simulink model "dyn_control"  (R2022a)
settings: Solver=VariableStepAuto  StartTime=0.0  StopTime=2  FixedStep=0.1  RelTol=1e-2
undefined symbols (not defined in the file): D, E_1, E_2, g, Gs_1, Gs_2, Ia_1, Ia_2, Im_1, Im_2, l_1, l_2, m_1, m_2, q_0, q_dot_0, t1_p, t2_p, t3_p, t4_p, t5_p, twt
libraries: slpidlib x2, matrix_library x2, dspinverses x2
settings Model: Creator=luca  LastModifiedBy=atled
settings SolverCC: AllowMultiTaskInputOutput=on  PositivePriorityOrder=on  AutoInsertRateTranBlk=on
settings HardwareCC: TargetBitPerPointer=64  TargetBitPerSizeT=64  TargetBitPerPtrDiffT=64  TargetLongLongMode=on  TargetIntDivRoundTo=Zero  TargetEndianess=LittleEndian  TargetWordSize=64  TargetHWDeviceType=MATLAB Host  ProdEqTarget=off
settings RTWCC: SystemTargetFile=raccel.tlc  TemplateMakefile=raccel_default_tmf  RTWVerbose=off
settings CodeAppCC: GenerateComments=off  MaxIdLength=128  SimulinkBlockComments=off
settings RaccelTargetCC: TargetLangStandard=C99 (ISO)  OptimizeReductions=off  ENABLE_SLEXEC_SSBRIDGE=1  RTWCAPISignals=off  RTWCAPIParams=off  RTWCAPIRootIO=off

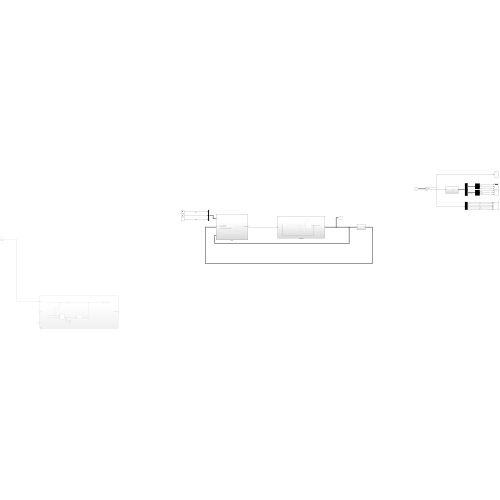
[thumbnail: Simulink's stored preview of the top-level diagram]
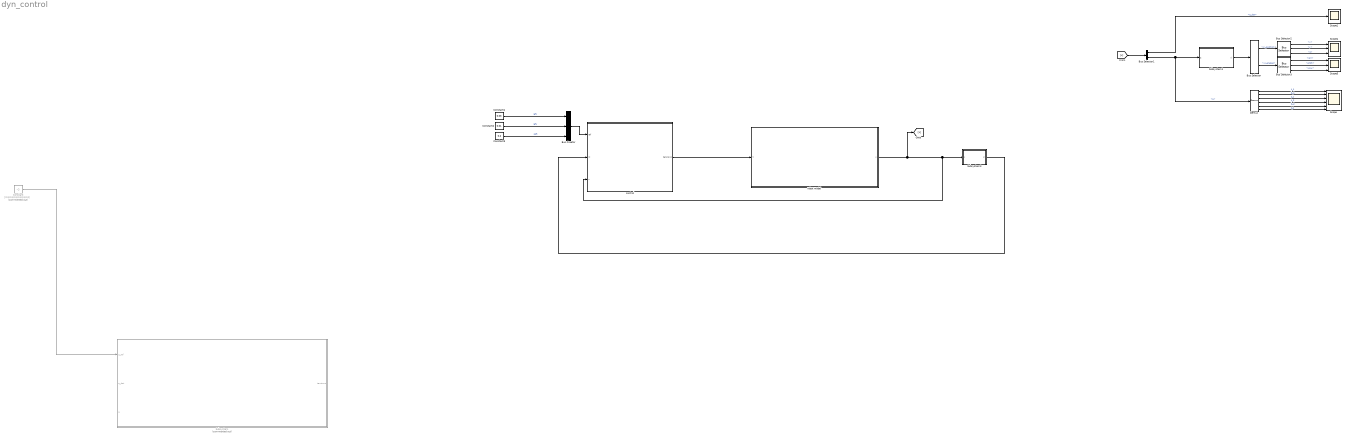
== system dyn_control ==
  Bus Creator : BusCreator  Inputs=3
  Bus Selector : BusSelector  OutputSignals=xi_position,xi_angles
  Bus Selector1 : BusSelector  OutputSignals=q_dot,q
  Bus Selector2 : BusSelector  OutputSignals=x,y,z
  Bus Selector3 : BusSelector  OutputSignals=roll,pitch,yaw
  Constant : Constant  Commented=on  Value=[0.3,0.3,0.3,0.3,0.3,0.3]
  Constant1 : Constant  Value=0.03  VectorParams1D=off
  Constant2 : Constant  Value=0.01  VectorParams1D=off
  Constant3 : Constant  Value=0.2  VectorParams1D=off
  Demux : Demux  Outputs=6
  Scope : Scope  NumInputPorts=6
  Scope1 : Scope
  Scope4 : Scope  NumInputPorts=3
  Scope5 : Scope  NumInputPorts=3
  Subsystem : Subsystem  Commented=on
  Subsystem1 : Subsystem
  Subsystem3 : Subsystem
  control : Subsystem
  robot model : Subsystem
  wires:
  Demux/1 -> Scope/1  "k_1"
  Demux/2 -> Scope/2  "b_1"
  Demux/3 -> Scope/3  "t_1"
  Demux/4 -> Scope/4  "k_2"
  Demux/5 -> Scope/5  "b_2"
  Demux/6 -> Scope/6  "t_2"
  Constant/1 -> Subsystem/1(q_ref)
  Subsystem1/1(xi) -> Bus Selector/1
  Bus Selector/1 -> Bus Selector2/1  "<xi_position>"
  Bus Selector/2 -> Bus Selector3/1  "<xi_angles>"
  [x] -> Bus Selector1/1
  Bus Selector1/2 -> Demux/1, Subsystem1/1(q)  "<q>"
  Bus Selector1/1 -> Scope1/1  "<q_dot>"
  Subsystem3/1(xi) -> control/2(Xi)
  robot model/1(x) -> [x], control/3(x), Subsystem3/1(x)
  Constant1/1 -> Bus Creator/1  "refx"
  Bus Selector2/1 -> Scope4/1  "<x>"
  Bus Selector2/2 -> Scope4/2  "<y>"
  Bus Selector2/3 -> Scope4/3  "<z>"
  Bus Selector3/1 -> Scope5/1  "<roll>"
  Bus Selector3/2 -> Scope5/2  "<pitch>"
  Bus Selector3/3 -> Scope5/3  "<yaw>"
  Constant2/1 -> Bus Creator/2  "refy"
  Constant3/1 -> Bus Creator/3  "refz"
  Bus Creator/1 -> control/1(ref)
  control/1(tensions) -> robot model/1(t)

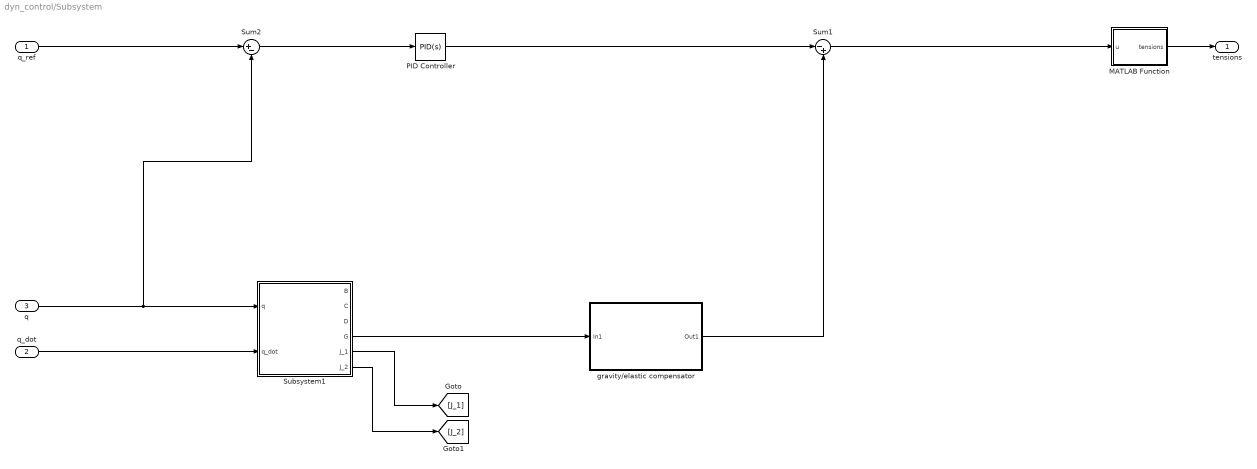
== system dyn_control/Subsystem ==
  q_ref : Inport
  q_dot : Inport  Port=2
  q : Inport  Port=3
  MATLAB Function : MATLAB Function  TreatAsAtomicUnit=on
  PID Controller : slpidlib/PID Controller  Controller=PID  Form=Parallel  TimeDomain=Continuous-time  UseExternalTs=off  SampleTime=-1  IntegratorMethod=Forward Euler  FilterMethod=Forward Euler  ControllerParametersSource=internal  P=1  I=0  UseKiTs=off  D=0.01  N=100  UseFilter=on  TunerSelectOption=Transfer Function Based (PID Tuner App)  InitialConditionSource=internal  InitialConditionForIntegrator=0  InitialConditionForFilter=0  DifferentiatorICPrevScaledInput=0  ExternalReset=none  TrackingMode=off  Kt=1  LimitOutput=off  SatLimitsSource=internal  UpperSaturationLimit=inf  LowerSaturationLimit=-inf  LinearizeAsGain=on  AntiWindupMode=none  Kb=1  POutMin=[]  POutMax=[]  IOutMin=[]  IOutMax=[]  DOutMin=[]  DOutMax=[]  NOutMin=[]  NOutMax=[]  SumOutMin=[]  SumOutMax=[]  SaturationOutMin=[]  SaturationOutMax=[]  PParamMin=[]  PParamMax=[]  IParamMin=[]  IParamMax=[]  DParamMin=[]  DParamMax=[]  NParamMin=[]  NParamMax=[]  KbParamMin=[]  KbParamMax=[]  KtParamMin=[]  KtParamMax=[]  KbOutMin=[]  KbOutMax=[]  KtOutMin=[]  KtOutMax=[]  IntegratorOutMin=[]  IntegratorOutMax=[]  FilterOutMin=[]  FilterOutMax=[]  SumI1OutMin=[]  SumI1OutMax=[]  SumI2OutMin=[]  SumI2OutMax=[]  SumI3OutMin=[]  SumI3OutMax=[]  SumI4OutMin=[]  SumI4OutMax=[]  SumDOutMin=[]  SumDOutMax=[]  DifferentiatorOutMin=[]  DifferentiatorOutMax=[]  FilterDiffOutCoefMin=[]  FilterDiffOutCoefMax=[]  ReciprocalOutMin=[]  ReciprocalOutMax=[]  SumDenOutMin=[]  SumDenOutMax=[]  SumNumOutMin=[]  SumNumOutMax=[]  DivideOutMin=[]  DivideOutMax=[]  UdiffTsProdOutMin=[]  UdiffTsProdOutMax=[]  NTsProdOutMin=[]  NTsProdOutMax=[]  UintegralTsProdOutMin=[]  UintegralTsProdOutMax=[]  UngainTsProdOutMin=[]  UngainTsProdOutMax=[]  IntegratorContinuousStateAttributes=''  IntegratorStateMustResolveToSignalObject=off  IntegratorRTWStateStorageClass=Auto  FilterContinuousStateAttributes=''  FilterStateMustResolveToSignalObject=off  FilterRTWStateStorageClass=Auto  ParallelPVariant=InternalParameters  IdealPVariant=Disabled  IVariant=InternalParameters  DVariant=InternalParameters  IntegratorVariant=Continuous  SatVariant=Disabled  AWVariant=Passthrough  PCopyVariant=Disabled  TRVariant=Disabled  FdbkBlocksVariant=Forward  IdealPFdbkVariant=Disabled  SatFdbkVariant=Disabled  DerivativeFilterVariant=ContFilter  NVariant=InternalParameters  NCopyVariant=Disabled  FilterICVariant=InternalICsFilter  IntegratorICVariant=InternalICs  ExternalResetVariant=Disabled  TRSumVariant=Passthrough  SumFdbkVariant=Disabled  SumVariant=Sum_PID  TsampFilterVariant=InternalTs  TsampNgainVariant=Passthrough  TsampIntegralVariant=Passthrough  ExternalSaturationOutDataTypeStr=Inherit: Same as second input  aMode=0
  Subsystem1 : Subsystem
  Sum1 : Sum  Inputs=|-+
  Sum2 : Sum  Inputs=|+-
  gravity/elastic compensator : Subsystem
  tensions : Outport
  wires:
  q/1 -> Subsystem1/1(q), Sum2/2
  q_dot/1 -> Subsystem1/2(q_dot)
  Subsystem1/4(G) -> gravity/elastic compensator/1(In1)
  gravity/elastic compensator/1(Out1) -> Sum1/2
  q_ref/1 -> Sum2/1
  PID Controller/1 -> Sum1/1
  Sum2/1 -> PID Controller/1
  Sum1/1 -> MATLAB Function/1(u)
  Subsystem1/5(J_1) -> [J_1]
  Subsystem1/6(J_2) -> [J_2]
  MATLAB Function/1(tensions) -> tensions/1

== system dyn_control/Subsystem1 ==
  q : Inport
  Bus Creator : BusCreator  Inputs=3
  Bus Creator1 : BusCreator  Inputs=2
  Bus Creator2 : BusCreator  Inputs=3
  Constant : Constant  Value=l_1
  Constant1 : Constant  Value=l_2
  MATLAB Function1 : MATLAB Function  TreatAsAtomicUnit=on
  xi : Outport
  wires:
  Constant1/1 -> MATLAB Function1/3(l_2)
  q/1 -> MATLAB Function1/1(q)
  Constant/1 -> MATLAB Function1/2(l_1)
  MATLAB Function1/1(x) -> Bus Creator/1  "x"
  MATLAB Function1/2(y) -> Bus Creator/2  "y"
  MATLAB Function1/3(z) -> Bus Creator/3  "z"
  MATLAB Function1/4(roll) -> Bus Creator2/1  "roll"
  MATLAB Function1/5(pitch) -> Bus Creator2/2  "pitch"
  MATLAB Function1/6(yaw) -> Bus Creator2/3  "yaw"
  Bus Creator/1 -> Bus Creator1/1  "xi_position"
  Bus Creator2/1 -> Bus Creator1/2  "xi_angles"
  Bus Creator1/1 -> xi/1

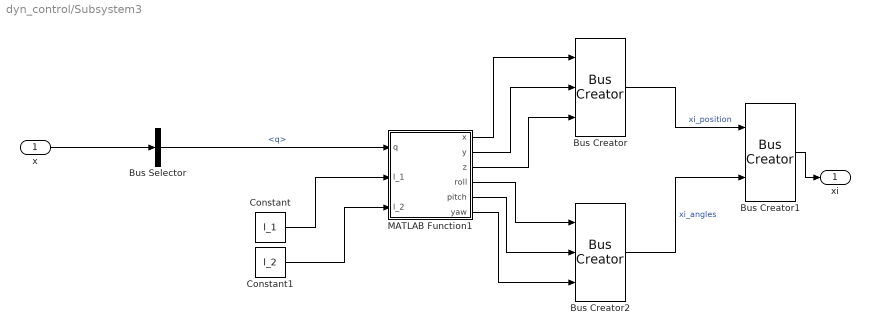
== system dyn_control/Subsystem3 ==
  x : Inport
  Bus Creator : BusCreator  Inputs=3
  Bus Creator1 : BusCreator  Inputs=2
  Bus Creator2 : BusCreator  Inputs=3
  Bus Selector : BusSelector  OutputSignals=q
  Constant : Constant  Value=l_1
  Constant1 : Constant  Value=l_2
  MATLAB Function1 : MATLAB Function  TreatAsAtomicUnit=on
  xi : Outport
  wires:
  Constant1/1 -> MATLAB Function1/3(l_2)
  Constant/1 -> MATLAB Function1/2(l_1)
  MATLAB Function1/1(x) -> Bus Creator/1
  MATLAB Function1/2(y) -> Bus Creator/2
  MATLAB Function1/3(z) -> Bus Creator/3
  MATLAB Function1/4(roll) -> Bus Creator2/1
  MATLAB Function1/5(pitch) -> Bus Creator2/2
  MATLAB Function1/6(yaw) -> Bus Creator2/3
  Bus Creator/1 -> Bus Creator1/1  "xi_position"
  Bus Creator2/1 -> Bus Creator1/2  "xi_angles"
  Bus Creator1/1 -> xi/1
  x/1 -> Bus Selector/1
  Bus Selector/1 -> MATLAB Function1/1(q)  "<q>"

== system dyn_control/control ==
  ref : Inport
  Xi : Inport  Port=2
  x : Inport  Port=3
  PD : Subsystem
      settings: PortSchema="{\"entries\":[{\"content\":{\"sides\":[{\"content\":{\"connectorIds\":[\"In1\",\"In2\"]},\"type\":\"ConnectorPlacement.EquallySpacedRectSide\",\"uuid\":\"ef742de7-f960-40b6-94f7-85e648a2417a\"},{\"content\":{\"connectorIds\":[\"Out1\"],\"side\":\"RIGHT\"},\"type\":\"ConnectorPlacement.EquallySpacedRectSide\",\"uuid\":\"e206da22-0c0c-407f-8f6d-88bececd3830\"},{\"content\":{\"connectorIds\":[],\"side\":\"TOP\"},\"type\":\"ConnectorPlacement.EquallySpacedRectSide\",\"uuid\":\"14c35c5b-992e-4e43-89c3-904fa34ec5bf\"},{\"content\":{\"connectorIds\":[\"In3\"],\"side\":\"BOTTOM\"},\"type\":\"ConnectorPlacement.EquallySpacedRectSide\",\"uuid\":\"998b2191-7e30-46d3-8883-46ecfd785cdd\"}]},\"type\":\"ConnectorPlacement.EquallySpacedConnector\",\"uuid\":\"de184336-5ab9-4a9a-8417-f4954e1c5ad0\"}],\"packageUris\":[\"http://schema.mathworks.com/mf0/Connector/R2020b\"],\"version\":\"1.0\"}"
  tensions : Outport
  wires:
  ref/1 -> PD/1(In1)
  Xi/1 -> PD/2(In2)
  x/1 -> PD/3(x)
  PD/1(t) -> tensions/1

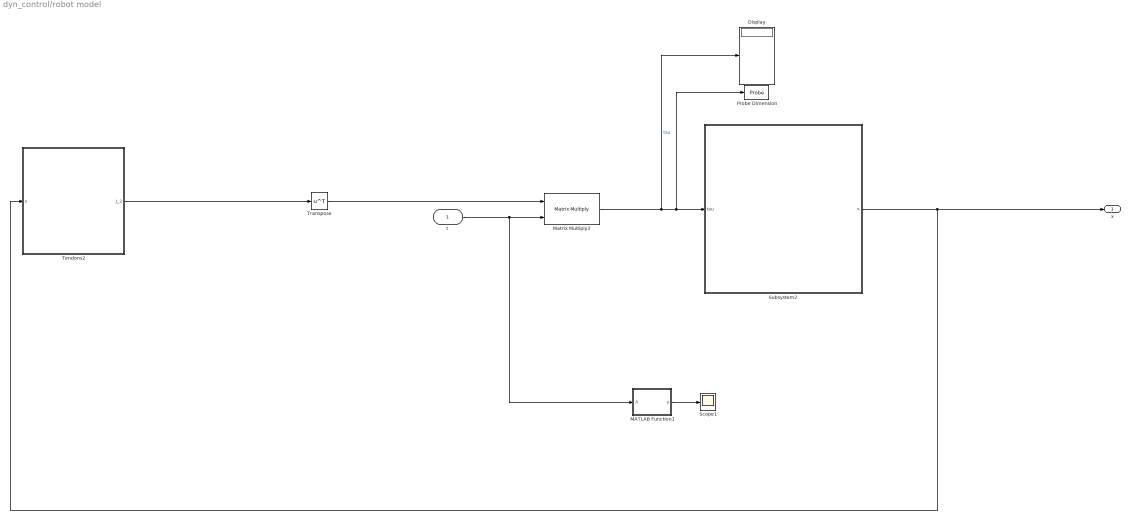
== system dyn_control/robot model ==
  t : Inport
  Display : Display
  MATLAB Function1 : MATLAB Function  TreatAsAtomicUnit=on
  Matrix Multiply3 : Product  Multiplication=Matrix(*)
  Probe Dimension : Probe  ProbeWidth=off  ProbeSampleTime=off  ProbeComplexSignal=off  ProbeSignalDimensions=on
  Scope1 : Scope
  Subsystem2 : Subsystem
  Tendons2 : Subsystem
  Transpose : Math  Operator=transpose
  x : Outport
  wires:
  Subsystem2/1(x) -> Tendons2/1(x), x/1
  Matrix Multiply3/1 -> Display/1, Probe Dimension/1, Subsystem2/1(tau)  "tau"
  Tendons2/1(J_2) -> Transpose/1
  Transpose/1 -> Matrix Multiply3/1
  t/1 -> MATLAB Function1/1(A), Matrix Multiply3/2
  MATLAB Function1/1(y) -> Scope1/1

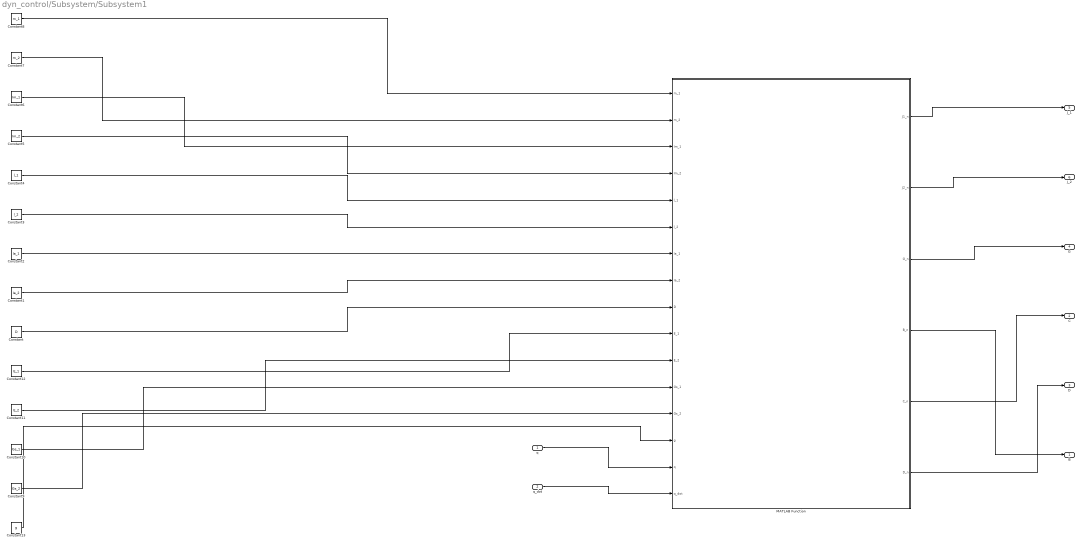
== system dyn_control/Subsystem/Subsystem1 ==
  q : Inport
  q_dot : Inport  Port=2
  Constant : Constant  Value=D
  Constant1 : Constant  Value=Ia_2
  Constant10 : Constant  Value=Gs_1
  Constant11 : Constant  Value=E_2
  Constant12 : Constant  Value=E_1
  Constant13 : Constant  Value=g
  Constant2 : Constant  Value=Ia_1
  Constant3 : Constant  Value=l_2
  Constant4 : Constant  Value=l_1
  Constant5 : Constant  Value=Im_2
  Constant6 : Constant  Value=Im_1
  Constant7 : Constant  Value=m_2
  Constant8 : Constant  Value=m_1
  Constant9 : Constant  Value=Gs_2
  MATLAB Function : MATLAB Function  TreatAsAtomicUnit=on
  B : Outport
  C : Outport  Port=2
  D : Outport  Port=3
  G : Outport  Port=4
  J_1 : Outport  Port=5
  J_2 : Outport  Port=6
  wires:
  MATLAB Function/1(J1_n) -> J_1/1
  MATLAB Function/3(G_n) -> G/1
  MATLAB Function/5(C_n) -> C/1
  MATLAB Function/2(J2_n) -> J_2/1
  MATLAB Function/4(B_n) -> B/1
  MATLAB Function/6(D_n) -> D/1
  q/1 -> MATLAB Function/15(q)
  q_dot/1 -> MATLAB Function/16(q_dot)
  Constant/1 -> MATLAB Function/9(D)
  Constant1/1 -> MATLAB Function/8(Ia_2)
  Constant2/1 -> MATLAB Function/7(Ia_1)
  Constant3/1 -> MATLAB Function/6(l_2)
  Constant4/1 -> MATLAB Function/5(l_1)
  Constant5/1 -> MATLAB Function/4(Im_2)
  Constant6/1 -> MATLAB Function/3(Im_1)
  Constant7/1 -> MATLAB Function/2(m_2)
  Constant8/1 -> MATLAB Function/1(m_1)
  Constant12/1 -> MATLAB Function/10(E_1)
  Constant11/1 -> MATLAB Function/11(E_2)
  Constant10/1 -> MATLAB Function/12(Gs_1)
  Constant9/1 -> MATLAB Function/13(Gs_2)
  Constant13/1 -> MATLAB Function/14(g)

== system dyn_control/Subsystem/gravity//elastic compensator ==
  In1 : Inport
  Constant : Constant  Value=0
  Manual Switch : ManualSwitch
  Out1 : Outport
  wires:
  Constant/1 -> Manual Switch/2
  Manual Switch/1 -> Out1/1
  In1/1 -> Manual Switch/1

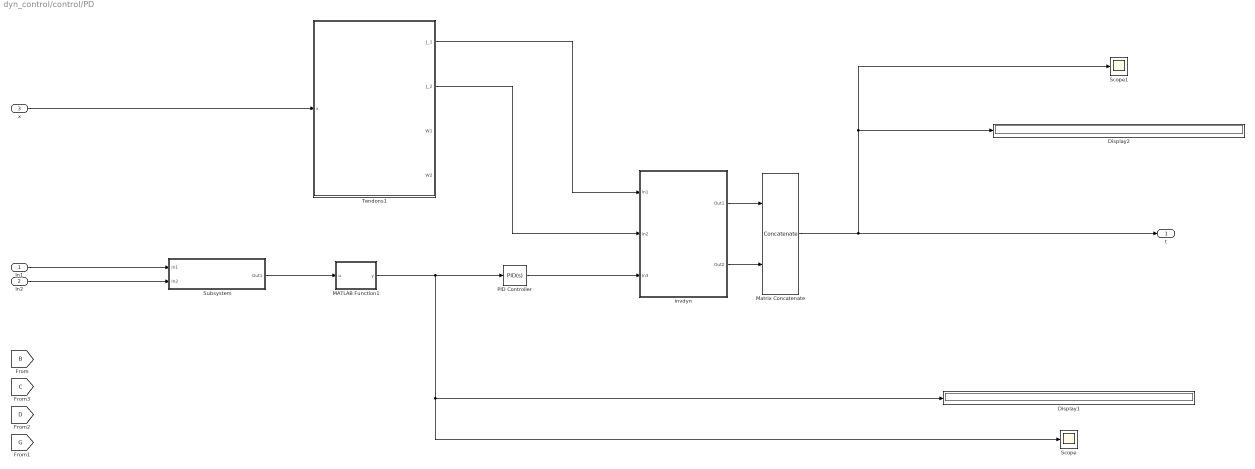
== system dyn_control/control/PD ==
  In1 : Inport
  In2 : Inport  Port=2
  x : Inport  Port=3
  Display1 : Display
  Display2 : Display
  MATLAB Function1 : MATLAB Function  TreatAsAtomicUnit=on
  Matrix Concatenate : Concatenate  Mode=Multidimensional array
  PID Controller : slpidlib/PID Controller  Controller=PID  Form=Parallel  TimeDomain=Continuous-time  UseExternalTs=off  SampleTime=-1  IntegratorMethod=Forward Euler  FilterMethod=Forward Euler  ControllerParametersSource=internal  P=[0,0,0,20,20,0]'  I=[0,0,0,0,0,0.1]'  UseKiTs=off  D=0.0001  N=100  UseFilter=on  TunerSelectOption=Transfer Function Based (PID Tuner App)  InitialConditionSource=internal  InitialConditionForIntegrator=0  InitialConditionForFilter=0  DifferentiatorICPrevScaledInput=0  ExternalReset=none  TrackingMode=off  Kt=1  LimitOutput=off  SatLimitsSource=internal  UpperSaturationLimit=inf  LowerSaturationLimit=-inf  LinearizeAsGain=on  AntiWindupMode=none  Kb=1  POutMin=[]  POutMax=[]  IOutMin=[]  IOutMax=[]  DOutMin=[]  DOutMax=[]  NOutMin=[]  NOutMax=[]  SumOutMin=[]  SumOutMax=[]  SaturationOutMin=[]  SaturationOutMax=[]  PParamMin=[]  PParamMax=[]  IParamMin=[]  IParamMax=[]  DParamMin=[]  DParamMax=[]  NParamMin=[]  NParamMax=[]  KbParamMin=[]  KbParamMax=[]  KtParamMin=[]  KtParamMax=[]  KbOutMin=[]  KbOutMax=[]  KtOutMin=[]  KtOutMax=[]  IntegratorOutMin=[]  IntegratorOutMax=[]  FilterOutMin=[]  FilterOutMax=[]  SumI1OutMin=[]  SumI1OutMax=[]  SumI2OutMin=[]  SumI2OutMax=[]  SumI3OutMin=[]  SumI3OutMax=[]  SumI4OutMin=[]  SumI4OutMax=[]  SumDOutMin=[]  SumDOutMax=[]  DifferentiatorOutMin=[]  DifferentiatorOutMax=[]  FilterDiffOutCoefMin=[]  FilterDiffOutCoefMax=[]  ReciprocalOutMin=[]  ReciprocalOutMax=[]  SumDenOutMin=[]  SumDenOutMax=[]  SumNumOutMin=[]  SumNumOutMax=[]  DivideOutMin=[]  DivideOutMax=[]  UdiffTsProdOutMin=[]  UdiffTsProdOutMax=[]  NTsProdOutMin=[]  NTsProdOutMax=[]  UintegralTsProdOutMin=[]  UintegralTsProdOutMax=[]  UngainTsProdOutMin=[]  UngainTsProdOutMax=[]  IntegratorContinuousStateAttributes=''  IntegratorStateMustResolveToSignalObject=off  IntegratorRTWStateStorageClass=Auto  FilterContinuousStateAttributes=''  FilterStateMustResolveToSignalObject=off  FilterRTWStateStorageClass=Auto  ParallelPVariant=InternalParameters  IdealPVariant=Disabled  IVariant=InternalParameters  DVariant=InternalParameters  IntegratorVariant=Continuous  SatVariant=Disabled  AWVariant=Passthrough  PCopyVariant=Disabled  TRVariant=Disabled  FdbkBlocksVariant=Forward  IdealPFdbkVariant=Disabled  SatFdbkVariant=Disabled  DerivativeFilterVariant=ContFilter  NVariant=InternalParameters  NCopyVariant=Disabled  FilterICVariant=InternalICsFilter  IntegratorICVariant=InternalICs  ExternalResetVariant=Disabled  TRSumVariant=Passthrough  SumFdbkVariant=Disabled  SumVariant=Sum_PID  TsampFilterVariant=InternalTs  TsampNgainVariant=Passthrough  TsampIntegralVariant=Passthrough  ExternalSaturationOutDataTypeStr=Inherit: Same as second input  aMode=0
  Scope : Scope
  Scope1 : Scope
  Subsystem : Subsystem
  Tendons1 : Subsystem
  invdyn : Subsystem
  t : Outport
  wires:
  MATLAB Function1/1(y) -> Display1/1, Scope/1, PID Controller/1
  Subsystem/1(Out1) -> MATLAB Function1/1(u)
  In2/1 -> Subsystem/2(In2)
  In1/1 -> Subsystem/1(In1)
  x/1 -> Tendons1/1(x)
  Matrix Concatenate/1 -> Display2/1, Scope1/1, t/1
  Tendons1/1(J_1) -> invdyn/1(In1)
  Tendons1/2(J_2) -> invdyn/2(In2)
  PID Controller/1 -> invdyn/3(In3)
  invdyn/1(Out1) -> Matrix Concatenate/1
  invdyn/2(Out2) -> Matrix Concatenate/2

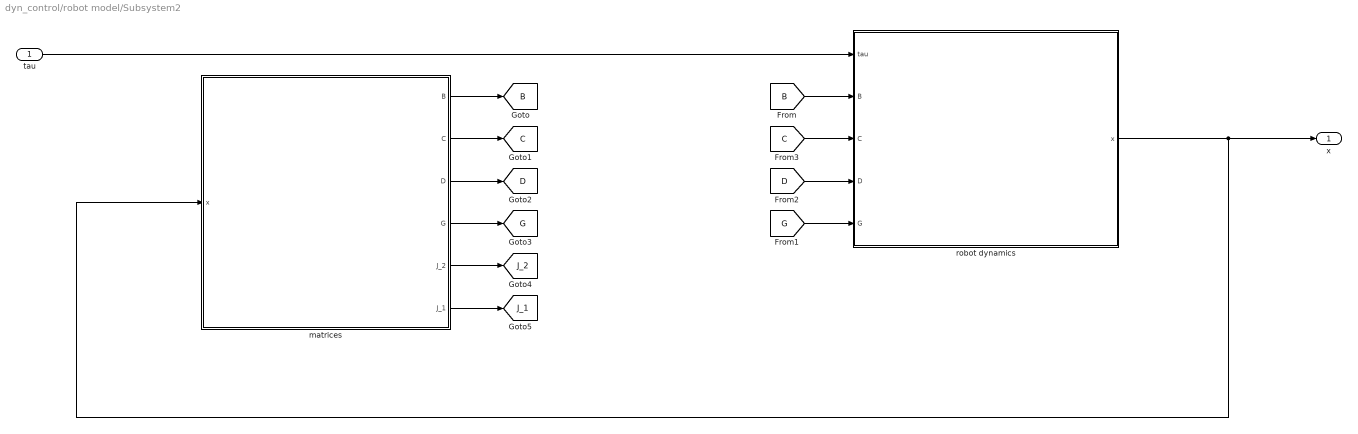
== system dyn_control/robot model/Subsystem2 ==
  tau : Inport
  matrices : Subsystem
  robot dynamics : Subsystem
  x : Outport
  tag scope: B=global, C=global, D=global, G=global, J_1=global, J_2=global
  wires:
  robot dynamics/1(x) -> matrices/1(x), x/1
  tau/1 -> robot dynamics/1(tau)
  matrices/1(B) -> [B]
  [B] -> robot dynamics/2(B)
  matrices/2(C) -> [C]
  matrices/3(D) -> [D]
  matrices/4(G) -> [G]
  [C] -> robot dynamics/3(C)
  [G] -> robot dynamics/5(G)
  [D] -> robot dynamics/4(D)
  matrices/5(J_2) -> [J_2]
  matrices/6(J_1) -> [J_1]

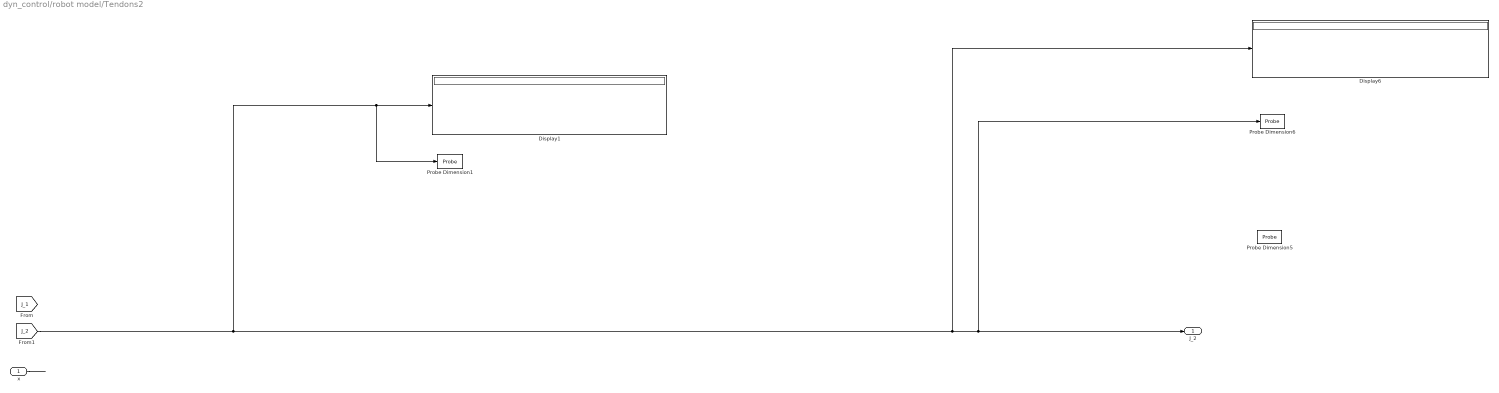
== system dyn_control/robot model/Tendons2 ==
  x : Inport
  Display1 : Display
  Display6 : Display
  Probe Dimension1 : Probe  ProbeWidth=off  ProbeSampleTime=off  ProbeComplexSignal=off  ProbeSignalDimensions=on
  Probe Dimension5 : Probe  ProbeWidth=off  ProbeSampleTime=off  ProbeComplexSignal=off  ProbeSignalDimensions=on
  Probe Dimension6 : Probe  ProbeWidth=off  ProbeSampleTime=off  ProbeComplexSignal=off  ProbeSignalDimensions=on
  J_2 : Outport
  wires:
  x/1 -> ?
  [J_2] -> J_2/1, Probe Dimension6/1, Display6/1, Probe Dimension1/1, Display1/1

== system dyn_control/control/PD/Subsystem ==
  In1 : Inport
  In2 : Inport  Port=2
  Bus Creator : BusCreator  Inputs=3
  Bus Selector : BusSelector  OutputSignals=refx,refy,refz
  Bus Selector1 : BusSelector  OutputSignals=xi_position.x,xi_position.y,xi_angles.yaw
  Sum1 : Sum  Inputs=|+-
  Sum2 : Sum  Inputs=|+-
  Sum3 : Sum  Inputs=|+-
  Out1 : Outport
  wires:
  Bus Selector1/3 -> Sum3/2  "<yaw>"
  Bus Selector/2 -> Sum2/1  "<refy>"
  In1/1 -> Bus Selector/1
  Sum1/1 -> Bus Creator/1
  Bus Selector1/2 -> Sum2/2  "<y>"
  Bus Selector/1 -> Sum1/1  "<refx>"
  Bus Selector/3 -> Sum3/1  "<refz>"
  Sum2/1 -> Bus Creator/2
  Sum3/1 -> Bus Creator/3
  Bus Selector1/1 -> Sum1/2  "<x>"
  Bus Creator/1 -> Out1/1
  In2/1 -> Bus Selector1/1

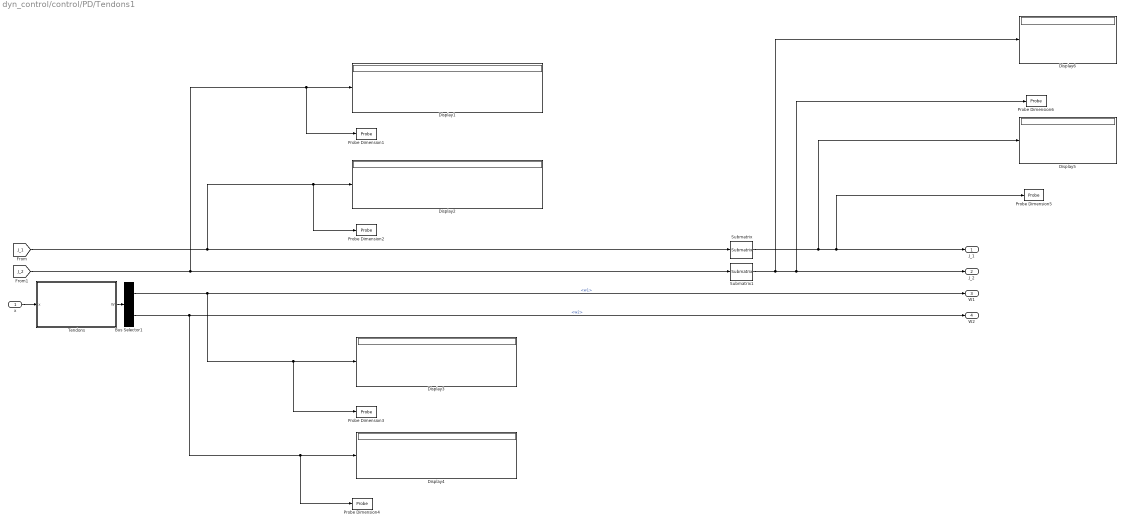
== system dyn_control/control/PD/Tendons1 ==
  x : Inport
  Bus Selector1 : BusSelector  OutputSignals=w1,w2
  Display{1..6} (6 alike) : Display
  Probe Dimension{1..6} (6 alike) : Probe  ProbeWidth=off  ProbeSampleTime=off  ProbeComplexSignal=off  ProbeSignalDimensions=on
  Submatrix : matrix_library/Submatrix  RowSpan=Range of rows  RowStartMode=Index  RowStartIndex=1  RowEndMode=Index  RowEndIndex=6  ColSpan=Range of columns  ColStartMode=Index  ColStartIndex=1  ColEndMode=Index  ColEndIndex=3
      settings: SourceProductBaseCode=SL
  Submatrix1 : matrix_library/Submatrix  RowSpan=Range of rows  RowStartMode=Index  RowStartIndex=1  RowEndMode=Index  RowEndIndex=6  ColSpan=Range of columns  ColStartMode=Index  ColStartIndex=1  ColEndMode=Index  ColEndIndex=3
      settings: SourceProductBaseCode=SL
  Tendons : Subsystem
  J_1 : Outport
  J_2 : Outport  Port=2
  W1 : Outport  Port=3
  W2 : Outport  Port=4
  wires:
  x/1 -> Tendons/1(x)
  Bus Selector1/2 -> Probe Dimension4/1, Display4/1, W2/1  "<w2>"
  Tendons/1(W) -> Bus Selector1/1
  Bus Selector1/1 -> Probe Dimension3/1, Display3/1, W1/1  "<w1>"
  [J_1] -> Submatrix/1, Probe Dimension2/1, Display2/1
  Submatrix/1 -> Display5/1, Probe Dimension5/1, J_1/1
  [J_2] -> Probe Dimension1/1, Display1/1, Submatrix1/1
  Submatrix1/1 -> J_2/1, Probe Dimension6/1, Display6/1

== system dyn_control/control/PD/invdyn ==
  In1 : Inport
  In2 : Inport  Port=2
  In3 : Inport  Port=3
  MatrixMultiply : Product  Multiplication=Matrix(*)
  MatrixMultiply1 : Product  Multiplication=Matrix(*)
  Pseudoinverse : dspinverses/Pseudoinverse  wanterr=off  SimulateUsing=Interpreted execution
      settings: SourceProductBaseCode=DS
  Pseudoinverse1 : dspinverses/Pseudoinverse  wanterr=off  SimulateUsing=Interpreted execution
      settings: SourceProductBaseCode=DS
  Out1 : Outport
  Out2 : Outport  Port=2
  wires:
  In3/1 -> MatrixMultiply/2, MatrixMultiply1/2
  In2/1 -> Pseudoinverse/1
  Pseudoinverse/1 -> MatrixMultiply/1
  In1/1 -> Pseudoinverse1/1
  Pseudoinverse1/1 -> MatrixMultiply1/1
  MatrixMultiply/1 -> Out2/1
  MatrixMultiply1/1 -> Out1/1

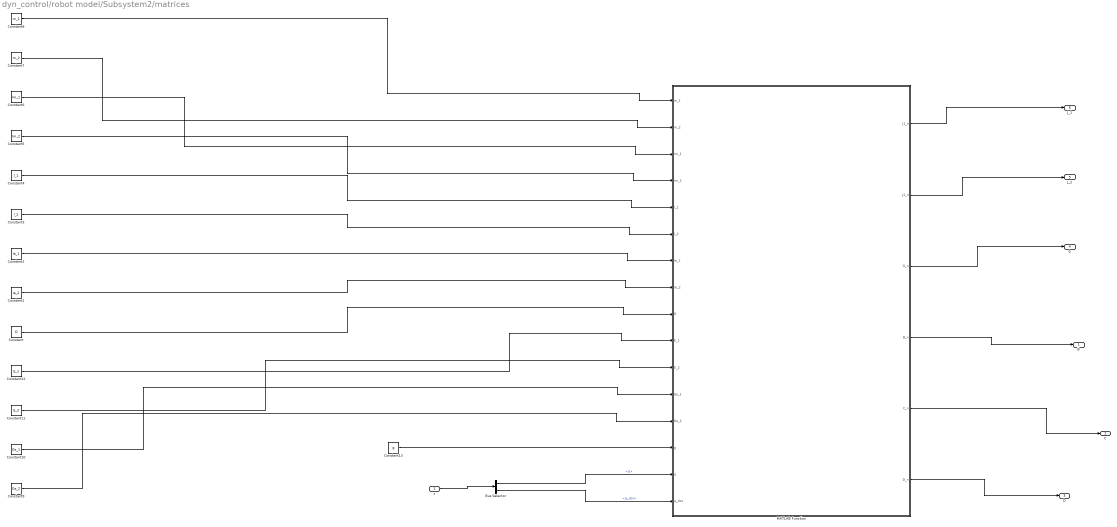
== system dyn_control/robot model/Subsystem2/matrices ==
  x : Inport
  Bus Selector : BusSelector  OutputSignals=q,q_dot
  Constant : Constant  Value=D
  Constant1 : Constant  Value=Ia_2
  Constant10 : Constant  Value=Gs_1
  Constant11 : Constant  Value=E_2
  Constant12 : Constant  Value=E_1
  Constant13 : Constant  Value=g
  Constant2 : Constant  Value=Ia_1
  Constant3 : Constant  Value=l_2
  Constant4 : Constant  Value=l_1
  Constant5 : Constant  Value=Im_2
  Constant6 : Constant  Value=Im_1
  Constant7 : Constant  Value=m_2
  Constant8 : Constant  Value=m_1
  Constant9 : Constant  Value=Gs_2
  MATLAB Function : MATLAB Function  TreatAsAtomicUnit=on
  B : Outport
  C : Outport  Port=2
  D : Outport  Port=3
  G : Outport  Port=4
  J_2 : Outport  Port=5
  J_1 : Outport  Port=6
  wires:
  MATLAB Function/1(J1_n) -> J_1/1
  MATLAB Function/3(G_n) -> G/1
  MATLAB Function/5(C_n) -> C/1
  MATLAB Function/2(J2_n) -> J_2/1
  MATLAB Function/4(B_n) -> B/1
  MATLAB Function/6(D_n) -> D/1
  Bus Selector/2 -> MATLAB Function/16(q_dot)  "<q_dot>"
  Constant/1 -> MATLAB Function/9(D)
  Constant1/1 -> MATLAB Function/8(Ia_2)
  Constant2/1 -> MATLAB Function/7(Ia_1)
  Constant3/1 -> MATLAB Function/6(l_2)
  Constant4/1 -> MATLAB Function/5(l_1)
  Constant5/1 -> MATLAB Function/4(Im_2)
  Constant6/1 -> MATLAB Function/3(Im_1)
  Constant7/1 -> MATLAB Function/2(m_2)
  Constant8/1 -> MATLAB Function/1(m_1)
  Constant12/1 -> MATLAB Function/10(E_1)
  Constant11/1 -> MATLAB Function/11(E_2)
  Constant10/1 -> MATLAB Function/12(Gs_1)
  Constant9/1 -> MATLAB Function/13(Gs_2)
  Constant13/1 -> MATLAB Function/14(g)
  Bus Selector/1 -> MATLAB Function/15(q)  "<q>"
  x/1 -> Bus Selector/1

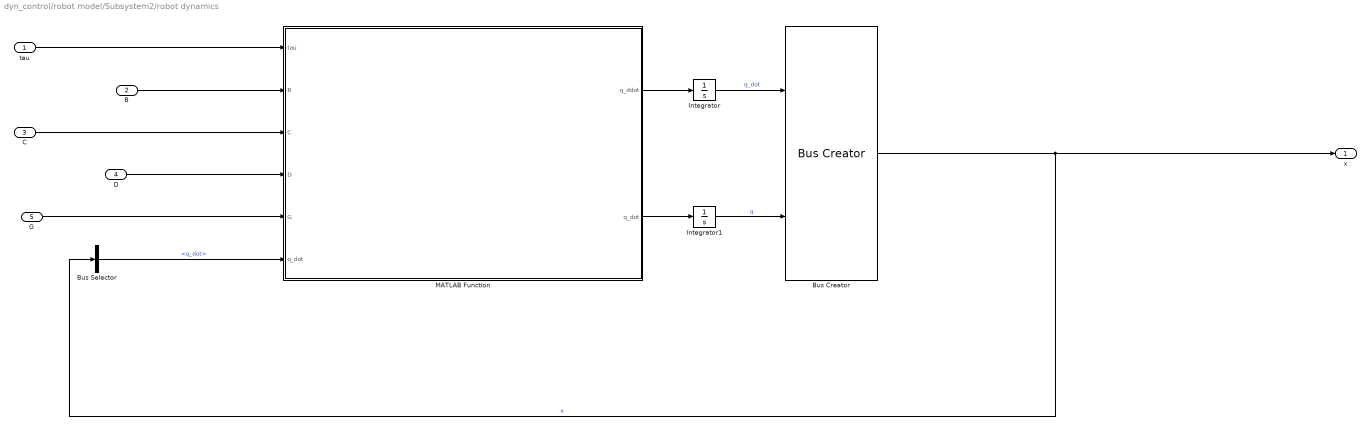
== system dyn_control/robot model/Subsystem2/robot dynamics ==
  tau : Inport
  B : Inport  Port=2
  C : Inport  Port=3
  D : Inport  Port=4
  G : Inport  Port=5
  Bus Creator : BusCreator  Inputs=2
  Bus Selector : BusSelector  OutputSignals=q_dot
  Integrator : Integrator  InitialCondition=q_dot_0
  Integrator1 : Integrator  InitialCondition=q_0
  MATLAB Function : MATLAB Function  TreatAsAtomicUnit=on
  x : Outport
  wires:
  Integrator/1 -> Bus Creator/1  "q_dot"
  MATLAB Function/1(q_ddot) -> Integrator/1
  B/1 -> MATLAB Function/2(B)
  C/1 -> MATLAB Function/3(C)
  D/1 -> MATLAB Function/4(D)
  G/1 -> MATLAB Function/5(G)
  MATLAB Function/2(q_dot) -> Integrator1/1
  Integrator1/1 -> Bus Creator/2  "q"
  Bus Selector/1 -> MATLAB Function/6("q_dot ")  "<q_dot>"
  Bus Creator/1 -> Bus Selector/1, x/1  "x"
  tau/1 -> MATLAB Function/1(tau)

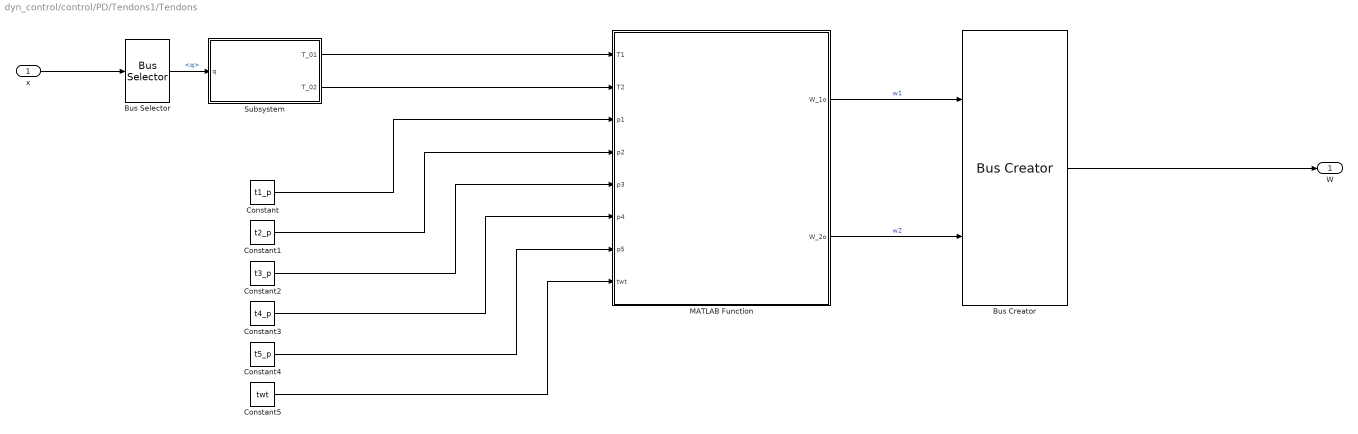
== system dyn_control/control/PD/Tendons1/Tendons ==
  x : Inport
  Bus Creator : BusCreator  Inputs=2
  Bus Selector : BusSelector  OutputSignals=q
  Constant : Constant  Value=t1_p
  Constant1 : Constant  Value=t2_p
  Constant2 : Constant  Value=t3_p
  Constant3 : Constant  Value=t4_p
  Constant4 : Constant  Value=t5_p
  Constant5 : Constant  Value=twt
  MATLAB Function : MATLAB Function  TreatAsAtomicUnit=on
  Subsystem : Subsystem
  W : Outport
  wires:
  MATLAB Function/2(W_2o) -> Bus Creator/2  "w2"
  MATLAB Function/1(W_1o) -> Bus Creator/1  "w1"
  Subsystem/1(T_01) -> MATLAB Function/1(T1)
  Subsystem/2(T_02) -> MATLAB Function/2(T2)
  Constant/1 -> MATLAB Function/3(p1)
  Constant1/1 -> MATLAB Function/4(p2)
  Constant2/1 -> MATLAB Function/5(p3)
  Constant3/1 -> MATLAB Function/6(p4)
  Constant4/1 -> MATLAB Function/7(p5)
  Constant5/1 -> MATLAB Function/8(twt)
  Bus Creator/1 -> W/1
  Bus Selector/1 -> Subsystem/1(q)  "<q>"
  x/1 -> Bus Selector/1

== system dyn_control/control/PD/Tendons1/Tendons/Subsystem ==
  q : Inport
  Constant : Constant  Value=l_1
  Constant1 : Constant  Value=l_2
  MATLAB Function1 : MATLAB Function  TreatAsAtomicUnit=on
  T_01 : Outport
  T_02 : Outport  Port=2
  wires:
  Constant1/1 -> MATLAB Function1/3(l_2)
  MATLAB Function1/2(T_02) -> T_02/1
  MATLAB Function1/1(T_01) -> T_01/1
  q/1 -> MATLAB Function1/1(q)
  Constant/1 -> MATLAB Function1/2(l_1)

== matlab function dyn_control/Subsystem3/MATLAB Function1 ==
  data: q input; x output; l_1 input; l_2 input; y output; z output; roll output; pitch output; yaw output
function [x , y , z , roll , pitch ,yaw ] = fcn(q,l_1,l_2)
    k_1 = q(1);
    b_1 = q(2);
    t_1 = q(3);
    k_2 = q(4);
    b_2 = q(5);
    t_2 = q(6);
    T1 = T_1(b_1,k_1,l_1,t_1);
    T2 = T_2(b_2,k_2,l_2,t_2);

    T_01 = T1;
    tw = T1 * T2;

    x = tw(1,4) ;
    y = tw(2,4) ;
    z = tw(3,4) ;
    roll = tw(3,2) ;
    pitch = tw(1,3) ;
    yaw = tw(2,1) ;

== matlab function dyn_control/robot model/Subsystem2/robot dynamics/MATLAB Function ==
  data: tau input; B input; C input; D input; G input; q_ddot output; q_dot input; q_dot output
function [ q_ddot,q_dot]  = fcn(tau,B,C,D,G,q_dot)
    q_dot = q_dot;
    q_ddot = - pinv(B) * ( G + ( C + D ) * q_dot - tau ) ;

== matlab function dyn_control/control/PD/MATLAB Function1 ==
  data: u input; y output
function y = fcn(u)
M = diag([1,0,0,0,0,0]);
y = [0 0 0 -u(2) -u(1) u(3)]'

== matlab function dyn_control/control/PD/Tendons1/Tendons/MATLAB Function ==
  data: T1 input; T2 input; p1 input; p2 input; p3 input; p4 input; p5 input; twt input; W_1o output; W_2o output
function [W_1o,W_2o] = fcn(T1,T2,p1,p2,p3, p4,p5,twt)

    %TENDON POSITION RESPECT (#0) BASE VERTEBRA CENTER
    T0_pos_1 = Ttr(p1);
    T0_pos_2 = Ttr(p2);
    T0_pos_3 = Ttr(p3);
    T0_pos_4 = Ttr(p4);
    T0_pos_5 = Tz(twt * 0) * Ttr(p5)  ;

    %TENDON POSITION RESPECT #1 VERTEBRA CENTER
    T1_pos_1 = Ttr(p1);
    T1_pos_2 = Ttr(p2);
    T1_pos_3 = Ttr(p3);
    T1_pos_4 = Ttr(p4);
    T1_pos_5 = Tz(twt * 1) * Ttr(p5)  ;
    
    %TENDON POSITION RESPECT #2 VERTEBRA CENTER
    T2_pos_1 = Ttr(p1);
    T2_pos_2 = Ttr(p2);
    T2_pos_3 = Ttr(p3);
    T2_pos_4 = Ttr(p4);
    T2_pos_5 = Tz(twt * 2) * Ttr(p5) ;

    %VERTEBRAE CENTER POSITION 
    O0 = eye(4);

    O0 = O0(1:3,4);
    O1 = T1(1:3,4);
    O2 = T2(1:3,4);

    %TENDON POSITION OF #0 (BASE) VERTEBRA RESPECT GLOBAL
    P_c01 = (T0_pos_1);
    P_c02 = (T0_pos_2);
    P_c03 = (T0_pos_3);
    P_c04 = (T0_pos_4);
    P_c05 = (T0_pos_5);

    P_cable_01 = P_c01(1:3,4);
    P_cable_02 = P_c02(1:3,4);
    P_cable_03 = P_c03(1:3,4);
    P_cable_04 = P_c04(1:3,4);
    P_cable_05 = P_c05(1:3,4);

    %TENDON POSITION OF #1 VERTEBRA RESPECT GLOBAL
    P_c11 = (T1 * T1_pos_1);
    P_c12 = (T1 * T1_pos_2);
    P_c13 = (T1 * T1_pos_3);
    P_c14 = (T1 * T1_pos_4);
    P_c15 = (T1 * T1_pos_5);

    P_cable_11 = P_c11(1:3,4);
    P_cable_12 = P_c12(1:3,4);
    P_cable_13 = P_c13(1:3,4);
    P_cable_14 = P_c14(1:3,4);
    P_cable_15 = P_c15(1:3,4);


    %TENDON POSITION OF #2 VERTEBRA RESPECT GLOBAL
    P_c21 = (T2 * T2_pos_1);
    P_c22 = (T2 * T2_pos_2);
    P_c23 = (T2 * T2_pos_3);
    P_c24 = (T2 * T2_pos_4);
    P_c25 = (T2 * T2_pos_5);

    P_cable_21 = P_c21(1:3,4);
    P_cable_22 = P_c22(1:3,4);
    P_cable_23 = P_c23(1:3,4);
    P_cable_24 = P_c24(1:3,4);
    P_cable_25 = P_c25(1:3,4);

    %WRENCH SECOND VERTEBRA
    
%     dp_1_1 = vectord(P_cable_11,P_cable_21);
%     dp_1_2 = vectord(P_cable_12,P_cable_22);
%     dp_1_3 = vectord(P_cable_13,P_cable_23);
%     dp_1_4 = vectord(P_cable_14,P_cable_24);
%     dp_1_5 = vectord(P_cable_15,P_cable_25);
%     
%     dp_O2_1 = vectord(O2,P_cable_21);
%     dp_O2_2 = vectord(O2,P_cable_22);
%     dp_O2_3 = vectord(O2,P_cable_23);
%     dp_O2_4 = vectord(O2,P_cable_24);
%     dp_O2_5 = vectord(O2,P_cable_25);
% 
%     dp_O1_1 = vectord(O1,P_cable_11);
%     dp_O1_2 = vectord(O1,P_cable_12);
%     dp_O1_3 = vectord(O1,P_cable_13);
%     dp_O1_4 = vectord(O1,P_cable_14);
%     dp_O1_5 = vectord(O1,P_cable_15);

%     F_2_1 = t(1) * dp_1_1 / norm(dp_1_1);
%     F_2_2 = t(2) * dp_1_2 / norm(dp_1_2);
%     F_2_3 = t(3) * dp_1_3 / norm(dp_1_3);
%     F_2_4 = t(4) * dp_1_4 / norm(dp_1_4);
%     F_2_5 = t(5) * dp_1_5 / norm(dp_1_5);
% 
%     M_2_1 = cross( dp_O2_1 , F_2_1);
%     M_2_2 = cross( dp_O2_2 , F_2_2);
%     M_2_3 = cross( dp_O2_3 , F_2_3);
%     M_2_4 = cross( dp_O2_4 , F_2_4);
%     M_2_5 = cross( dp_O2_5 , F_2_5);
% 
%     F_2 = F_2_1 + F_2_2 + F_2_3 + F_2_4 + F_2_5 ;
%     
%     M_2 = M_2_1 + M_2_2 + M_2_3 + M_2_4 + M_2_5 + cross( vectord(O1,O2) , F_2);
%     
%     %WRENCH FIRST VERTEBRA
%     dp_2_1 = vectord(P_cable_21,P_cable_11);
%     dp_2_2 = vectord(P_cable_22,P_cable_12);
%     dp_2_3 = vectord(P_cable_23,P_cable_13);
%     dp_2_4 = vectord(P_cable_24,P_cable_14);
%     dp_2_5 = vectord(P_cable_25,P_cable_15);
%    
%     dp_0_1 = vectord(P_cable_01,P_cable_11);
%     dp_0_2 = vectord(P_cable_02,P_cable_12);
%     dp_0_3 = vectord(P_cable_03,P_cable_13);
%     dp_0_4 = vectord(P_cable_04,P_cable_14);
%     dp_0_5 = vectord(P_cable_05,P_cable_15);
% 
%     F_1_1 = t(1) * dp_2_1 / norm(dp_2_1) + t(1) * dp_0_1 / norm(dp_0_1);
%     F_1_2 = t(2) * dp_2_2 / norm(dp_2_2) + t(2) * dp_0_2 / norm(dp_0_2);
%     F_1_3 = t(3) * dp_2_3 / norm(dp_2_3) + t(3) * dp_0_3 / norm(dp_0_3);
%     F_1_4 = t(4) * dp_2_4 / norm(dp_2_4) + t(4) * dp_0_4 / norm(dp_0_4);
%     F_1_5 = t(5) * dp_2_5 / norm(dp_2_5) + t(5) * dp_0_5 / norm(dp_0_5);
% 
%     F_1 = F_1_1 + F_1_2 + F_1_3 + F_1_4 + F_1_5 + F_2;
% 
%     M_1_1 = cross( dp_O1_1 , F_1_1);
%     M_1_2 = cross( dp_O1_2 , F_1_2);
%     M_1_3 = cross( dp_O1_3 , F_1_3);
%     M_1_4 = cross( dp_O1_4 , F_1_4);
%     M_1_5 = cross( dp_O1_5 , F_1_5);
% 
%     M_1 = M_1_1 + M_1_2 + M_1_3 + M_1_4 + M_1_5 + cross( vectord(O0,O1) , F_1) + M_2;
% 
%     w1 = [ F_1' , M_1' ]';
%     w2 = [ F_2' , M_2' ]';

    %MATRICES
    W_1 = zeros(6,5);
    W_2 = zeros(6,5);

    W_2(1:3,1) = compute_force_final(P_cable_21,P_cable_11);
    W_2(1:3,2) = compute_force_final(P_cable_22,P_cable_12);
    W_2(1:3,3) = compute_force_final(P_cable_23,P_cable_13);
    W_2(1:3,4) = compute_force_final(P_cable_24,P_cable_14);
    W_2(1:3,5) = compute_force_final(P_cable_25,P_cable_15);


    W_2(4:6,1) = compute_momentum_final(P_cable_21,P_cable_11,O2) + cross( vectord(O1,O2) , W_2(1:3,1) ) ;
    W_2(4:6,2) = compute_momentum_final(P_cable_22,P_cable_12,O2) + cross( vectord(O1,O2) , W_2(1:3,2) ) ;
    W_2(4:6,3) = compute_momentum_final(P_cable_23,P_cable_13,O2) + cross( vectord(O1,O2) , W_2(1:3,3) ) ;
    W_2(4:6,4) = compute_momentum_final(P_cable_24,P_cable_14,O2) + cross( vectord(O1,O2) , W_2(1:3,4) ) ;
    W_2(4:6,5) = compute_momentum_final(P_cable_25,P_cable_15,O2) + cross( vectord(O1,O2) , W_2(1:3,5) ) ;


    W_1(1:3,1) = compute_force_middle(P_cable_11,P_cable_01,P_cable_21) + W_2(1:3,1);
    W_1(1:3,2) = compute_force_middle(P_cable_12,P_cable_02,P_cable_22) + W_2(1:3,2);
    W_1(1:3,3) = compute_force_middle(P_cable_13,P_cable_03,P_cable_23) + W_2(1:3,3);
    W_1(1:3,4) = compute_force_middle(P_cable_14,P_cable_04,P_cable_24) + W_2(1:3,4);
    W_1(1:3,5) = compute_force_middle(P_cable_15,P_cable_05,P_cable_25) + W_2(1:3,5);

    W_1(4:6,1) = compute_momentum_middle(P_cable_11,P_cable_01,P_cable_21,O1) + W_2(4:6,1) + cross( vectord(O0,O1) , W_1(1:3,1)) ;
    W_1(4:6,2) = compute_momentum_middle(P_cable_12,P_cable_02,P_cable_22,O1) + W_2(4:6,2) + cross( vectord(O0,O1) , W_1(1:3,2)) ;
    W_1(4:6,3) = compute_momentum_middle(P_cable_13,P_cable_03,P_cable_23,O1) + W_2(4:6,3) + cross( vectord(O0,O1) , W_1(1:3,3)) ;
    W_1(4:6,4) = compute_momentum_middle(P_cable_14,P_cable_04,P_cable_24,O1) + W_2(4:6,4) + cross( vectord(O0,O1) , W_1(1:3,4)) ;
    W_1(4:6,5) = compute_momentum_middle(P_cable_15,P_cable_05,P_cable_25,O1) + W_2(4:6,5) + cross( vectord(O0,O1) , W_1(1:3,5)) ;

    W_1o = W_1;
    W_2o = W_2;


    function n = compute_direction(p1) 
        n = p1 / norm(p1);
    end 

    function F = compute_force_final(pkn,pknm1) 
        dp = vectord(pkn,pknm1);
        F = compute_direction(dp);
    end 

    function F = compute_force_middle(pkj,pkjm1,pkjp1) 
        dpm = vectord(pkj,pkjm1);
        dpp = vectord(pkj,pkjp1);
        F = compute_direction(dpm) - compute_direction(dpp);
    end 

    function M = compute_momentum_middle(pkj,pkjm1,pkjp1,Oj) 
        F = compute_force_middle(pkj,pkjm1,pkjp1);
        M = cross( vectord(Oj,pkj) , F );
    end

    function M = compute_momentum_final(pkn,pknm1,On) 
        F = compute_force_final(pkn,pknm1) ;
        M = cross( vectord(On,pkn) , F );
    end 
end

== matlab function dyn_control/robot model/MATLAB Function1 ==
  data: A input; y output
function y = fcn(A)
 y = cond(A)

== matlab function dyn_control/control/PD/Tendons1/Tendons/Subsystem/MATLAB Function1 ==
  data: q input; T_01 output; T_02 output; l_1 input; l_2 input
function [T_01,T_02] = fcn(q,l_1,l_2)
    k_1 = q(1);
    b_1 = q(2);
    t_1 = q(3);
    k_2 = q(4);
    b_2 = q(5);
    t_2 = q(6);
    T1 = T_1(b_1,k_1,l_1,t_1);
    T2 = T_2(b_2,k_2,l_2,t_2);

    T_01 = T1;
    T_02 = T1 * T2;

== matlab function dyn_control/Subsystem/Subsystem1/MATLAB Function ==
  data: m_1 input; J1_n output; J2_n output; G_n output; B_n output; C_n output; D_n output; m_2 input; Im_1 input; Im_2 input; l_1 input; l_2 input; Ia_1 input; Ia_2 input; D input; E_1 input; E_2 input; Gs_1 input; Gs_2 input; g input; q input; q_dot input
function [J1_n,J2_n,G_n,B_n,C_n,D_n] = DYNAMIC_MATRICES(m_1,m_2,Im_1,Im_2,l_1,l_2,Ia_1,Ia_2,D,E_1,E_2,Gs_1,Gs_2,g,q,q_dot)

k_1 = q(1);
b_1 = q(2);
t_1 = q(3);
k_2 = q(4);
b_2 = q(5);
t_2 = q(6);

k_dot_1 = q_dot(1);
b_dot_1 = q_dot(2);
t_dot_1 = q_dot(3);
k_dot_2 = q_dot(4);
b_dot_2 = q_dot(5);
t_dot_2 = q_dot(6);

Iax_1 = Ia_1(1,1);
Iay_1 = Ia_1(2,2);
Iaz_1 = Ia_1(3,3);

Iax_2 = Ia_2(1,1);
Iay_2 = Ia_2(2,2);
Iaz_2 = Ia_2(3,3);

Imx_1 = Im_1(1,1);
Imy_1 = Im_1(2,2);
Imz_1 = Im_1(3,3);

Imx_2 = Im_2(1,1);
Imy_2 = Im_2(2,2);
Imz_2 = Im_2(3,3);


g_x = g(1);
g_y = g(2);
g_z = g(3);

C_1_1 = C11(Imx_1,Imx_2,Imy_1,Imy_2,Imz_1,Imz_2,b_1,b_2,b_dot_1,b_dot_2,k_1,k_2,k_dot_1,k_dot_2,l_1,l_2,m_1,m_2,t_1,t_2,t_dot_1,t_dot_2);
C_1_2 = C12(Imx_1,Imx_2,Imy_1,Imy_2,Imz_1,Imz_2,b_1,b_2,b_dot_1,b_dot_2,k_1,k_2,k_dot_1,k_dot_2,l_1,l_2,m_1,m_2,t_1,t_2,t_dot_1,t_dot_2);
C_1_3 = C13(Imx_1,Imx_2,Imy_1,Imy_2,Imz_1,Imz_2,b_1,b_2,b_dot_1,b_dot_2,k_1,k_2,k_dot_1,k_dot_2,l_1,l_2,m_1,m_2,t_1,t_2,t_dot_1,t_dot_2);
C_1_4 = C14(Imx_2,Imy_2,Imz_2,b_1,b_2,b_dot_1,b_dot_2,k_1,k_2,k_dot_1,k_dot_2,l_1,l_2,m_2,t_1,t_2,t_dot_1,t_dot_2);
C_1_5 = C15(Imx_2,Imy_2,Imz_2,b_1,b_2,b_dot_1,b_dot_2,k_1,k_2,k_dot_1,k_dot_2,l_1,l_2,m_2,t_1,t_2,t_dot_1,t_dot_2);
C_1_6 = C16(Imx_2,Imy_2,Imz_2,b_1,b_2,b_dot_1,b_dot_2,k_1,k_2,k_dot_1,k_dot_2,l_1,l_2,m_2,t_1,t_2,t_dot_1,t_dot_2);

C_2_1 = C21(Imx_1,Imx_2,Imy_1,Imy_2,Imz_1,Imz_2,b_1,b_2,b_dot_1,b_dot_2,k_1,k_2,k_dot_1,k_dot_2,l_1,l_2,m_1,m_2,t_1,t_2,t_dot_1,t_dot_2);
C_2_2 = C21(Imx_1,Imx_2,Imy_1,Imy_2,Imz_1,Imz_2,b_1,b_2,b_dot_1,b_dot_2,k_1,k_2,k_dot_1,k_dot_2,l_1,l_2,m_1,m_2,t_1,t_2,t_dot_1,t_dot_2);
C_2_3 = C21(Imx_1,Imx_2,Imy_1,Imy_2,Imz_1,Imz_2,b_1,b_2,b_dot_1,b_dot_2,k_1,k_2,k_dot_1,k_dot_2,l_1,l_2,m_1,m_2,t_1,t_2,t_dot_1,t_dot_2);
C_2_4 = C26(Imx_2,Imy_2,Imz_2,b_1,b_2,b_dot_1,b_dot_2,k_1,k_2,k_dot_1,k_dot_2,l_1,l_2,m_2,t_1,t_2,t_dot_1,t_dot_2);
C_2_5 = C26(Imx_2,Imy_2,Imz_2,b_1,b_2,b_dot_1,b_dot_2,k_1,k_2,k_dot_1,k_dot_2,l_1,l_2,m_2,t_1,t_2,t_dot_1,t_dot_2);
C_2_6 = C26(Imx_2,Imy_2,Imz_2,b_1,b_2,b_dot_1,b_dot_2,k_1,k_2,k_dot_1,k_dot_2,l_1,l_2,m_2,t_1,t_2,t_dot_1,t_dot_2);

C_3_1 = C31(Imx_1,Imx_2,Imy_1,Imy_2,Imz_1,Imz_2,b_1,b_2,b_dot_1,b_dot_2,k_1,k_2,k_dot_1,k_dot_2,l_1,l_2,m_1,m_2,t_1,t_2,t_dot_1,t_dot_2);
C_3_2 = C32(Imx_1,Imx_2,Imy_1,Imy_2,Imz_1,Imz_2,b_1,b_2,b_dot_1,b_dot_2,k_1,k_2,k_dot_1,k_dot_2,l_1,l_2,m_1,m_2,t_1,t_2,t_dot_1,t_dot_2);
C_3_3 = C33(Imx_1,Imx_2,Imy_1,Imy_2,Imz_1,Imz_2,b_1,b_2,b_dot_1,b_dot_2,k_1,k_2,k_dot_1,k_dot_2,l_1,l_2,m_1,m_2,t_1,t_2,t_dot_1,t_dot_2);
C_3_4 =C34(Imx_2,Imy_2,Imz_2,b_1,b_2,b_dot_1,b_dot_2,k_1,k_2,k_dot_1,k_dot_2,l_1,l_2,m_2,t_1,t_2,t_dot_1,t_dot_2);
C_3_5 = C35(Imx_2,Imy_2,Imz_2,b_1,b_2,b_dot_1,b_dot_2,k_1,k_2,k_dot_1,k_dot_2,l_1,l_2,m_2,t_1,t_2,t_dot_1,t_dot_2);
C_3_6 =C36(Imx_2,Imy_2,Imz_2,b_1,b_2,b_dot_1,b_dot_2,k_1,k_2,k_dot_1,k_dot_2,l_1,l_2,m_2,t_1,t_2,t_dot_1,t_dot_2);

C_4_1 = C41(Imx_2,Imy_2,Imz_2,b_1,b_2,b_dot_1,b_dot_2,k_1,k_2,k_dot_1,k_dot_2,l_1,l_2,m_2,t_1,t_2,t_dot_1,t_dot_2);
C_4_2 = C42(Imx_2,Imy_2,Imz_2,b_1,b_2,b_dot_1,b_dot_2,k_1,k_2,k_dot_1,k_dot_2,l_1,l_2,m_2,t_1,t_2,t_dot_1,t_dot_2);
C_4_3 =C43(Imx_2,Imy_2,Imz_2,b_1,b_2,b_dot_1,b_dot_2,k_1,k_2,k_dot_1,k_dot_2,l_1,l_2,m_2,t_1,t_2,t_dot_1,t_dot_2);
C_4_4 =C44(Imx_2,Imy_2,Imz_2,b_1,b_2,b_dot_1,b_dot_2,k_1,k_2,k_dot_1,k_dot_2,l_1,l_2,m_2,t_1,t_2,t_dot_1,t_dot_2);
C_4_5 =C45(Imx_2,Imy_2,Imz_2,b_1,b_2,b_dot_1,b_dot_2,k_1,k_2,k_dot_1,k_dot_2,l_1,l_2,m_2,t_1,t_2,t_dot_1,t_dot_2);
C_4_6 =C46(Imx_2,Imy_2,Imz_2,b_1,b_2,b_dot_1,b_dot_2,k_1,k_2,k_dot_1,k_dot_2,l_1,l_2,m_2,t_1,t_2,t_dot_1,t_dot_2);

C_5_1 =C51(Imx_2,Imy_2,Imz_2,b_1,b_2,b_dot_1,b_dot_2,k_1,k_2,k_dot_1,k_dot_2,l_1,l_2,m_2,t_1,t_2,t_dot_1,t_dot_2);
C_5_2 = C52(Imx_2,Imy_2,Imz_2,b_1,b_2,b_dot_1,b_dot_2,k_1,k_2,k_dot_1,k_dot_2,l_1,l_2,m_2,t_1,t_2,t_dot_1,t_dot_2);
C_5_3 =C53(Imx_2,Imy_2,Imz_2,b_1,b_2,b_dot_1,b_dot_2,k_1,k_2,k_dot_1,k_dot_2,l_1,l_2,m_2,t_1,t_2,t_dot_1,t_dot_2);
C_5_4 =C54(Imx_2,Imy_2,Imz_2,b_1,b_2,b_dot_1,b_dot_2,k_1,k_2,k_dot_1,k_dot_2,l_1,l_2,m_2,t_1,t_2,t_dot_1,t_dot_2);
C_5_5 =C55(Imx_2,Imy_2,Imz_2,b_1,b_2,b_dot_1,b_dot_2,k_1,k_2,k_dot_1,k_dot_2,l_1,l_2,m_2,t_1,t_2,t_dot_1,t_dot_2);
C_5_6 =C56(Imx_2,Imy_2,Imz_2,b_1,b_2,b_dot_1,b_dot_2,k_1,k_2,k_dot_1,k_dot_2,l_1,l_2,m_2,t_1,t_2,t_dot_1,t_dot_2);

C_6_1 =C61(Imx_2,Imy_2,Imz_2,b_1,b_2,b_dot_1,b_dot_2,k_1,k_2,k_dot_1,k_dot_2,l_1,l_2,m_2,t_1,t_2,t_dot_1,t_dot_2);
C_6_2 = C62(Imx_2,Imy_2,Imz_2,b_1,b_2,b_dot_1,b_dot_2,k_1,k_2,k_dot_1,k_dot_2,l_1,l_2,m_2,t_1,t_2,t_dot_1,t_dot_2);
C_6_3 =C63(Imx_2,Imy_2,Imz_2,b_1,b_2,b_dot_1,b_dot_2,k_1,k_2,k_dot_1,k_dot_2,l_1,l_2,m_2,t_1,t_2,t_dot_1,t_dot_2);
C_6_4 =C64(Imx_2,Imy_2,Imz_2,b_1,b_2,b_dot_1,b_dot_2,k_1,k_2,k_dot_1,k_dot_2,l_1,l_2,m_2,t_1,t_2,t_dot_1,t_dot_2);
C_6_5 =C65(Imx_2,Imy_2,Imz_2,b_1,b_2,b_dot_1,b_dot_2,k_1,k_2,k_dot_1,k_dot_2,l_1,l_2,m_2,t_1,t_2,t_dot_1,t_dot_2);
C_6_6 =C66(Imx_2,Imy_2,Imz_2,b_1,b_2,b_dot_1,b_dot_2,k_1,k_2,k_dot_1,k_dot_2,l_1,l_2,m_2,t_1,t_2,t_dot_1,t_dot_2);

C_n = [ C_1_1,C_1_2,C_1_3,C_1_4,C_1_5,C_1_6;
        C_2_1,C_2_2,C_2_3,C_2_4,C_2_5,C_2_6;
        C_3_1,C_3_2,C_3_3,C_3_4,C_3_5,C_3_6;
        C_4_1,C_4_2,C_4_3,C_4_4,C_4_5,C_4_6;
        C_5_1,C_5_2,C_5_3,C_5_4,C_5_5,C_5_6;
        C_6_1,C_6_2,C_6_3,C_6_4,C_6_5,C_6_6;
      ];
 J1_n= J_1(b_1,k_1,l_1,t_1);
 J2_n= J_2(b_1,b_2,k_1,k_2,l_1,l_2,t_1,t_2);
 B_n=B(Imx_1,Imx_2,Imy_1,Imy_2,Imz_1,Imz_2,b_1,b_2,k_1,k_2,l_1,l_2,m_1,m_2,t_1,t_2);
 G_n =G(E_1,E_2,Gs_1,Gs_2,Iax_1,Iax_2,Iay_1,Iay_2,Iaz_1,Iaz_2,b_1,b_2,g_x,g_y,g_z,k_1,k_2,l_1,l_2,m_1,m_2,t_1,t_2);
D_n = D;

== matlab function dyn_control/robot model/Subsystem2/matrices/MATLAB Function ==
  data: m_1 input; J1_n output; J2_n output; G_n output; B_n output; C_n output; D_n output; m_2 input; Im_1 input; Im_2 input; l_1 input; l_2 input; Ia_1 input; Ia_2 input; D input; E_1 input; E_2 input; Gs_1 input; Gs_2 input; g input; q input; q_dot input
function [J1_n,J2_n,G_n,B_n,C_n,D_n] = dynamics_matrices(m_1,m_2,Im_1,Im_2,l_1,l_2,Ia_1,Ia_2,D,E_1,E_2,Gs_1,Gs_2,g,q,q_dot)

k_1 = q(1);
b_1 = q(2);
t_1 = q(3);
k_2 = q(4);
b_2 = q(5);
t_2 = q(6);

k_dot_1 = q_dot(1);
b_dot_1 = q_dot(2);
t_dot_1 = q_dot(3);
k_dot_2 = q_dot(4);
b_dot_2 = q_dot(5);
t_dot_2 = q_dot(6);

Iax_1 = Ia_1(1,1);
Iay_1 = Ia_1(2,2);
Iaz_1 = Ia_1(3,3);

Iax_2 = Ia_2(1,1);
Iay_2 = Ia_2(2,2);
Iaz_2 = Ia_2(3,3);

Imx_1 = Im_1(1,1);
Imy_1 = Im_1(2,2);
Imz_1 = Im_1(3,3);

Imx_2 = Im_2(1,1);
Imy_2 = Im_2(2,2);
Imz_2 = Im_2(3,3);

A = 0;
A_2 = 0;

g_x = g(1);
g_y = g(2);
g_z = g(3);

C_1_1 = C11(k_1,b_1,t_1,k_2,b_2,t_2,k_dot_1,b_dot_1,t_dot_1,k_dot_2,b_dot_2,t_dot_2,l_1,l_2,A,A_2,Iax_2,Iay_2,Iaz_2,Iax_1,Iay_1,Iaz_1,Imx_1,Imy_1,Imz_1,Imx_2,Imy_2,Imz_2,m_1,m_2,g_x,g_y,g_z,Gs_1,E_1,Gs_2,E_2);
C_1_2 = C12(k_1,b_1,t_1,k_2,b_2,t_2,k_dot_1,b_dot_1,t_dot_1,k_dot_2,b_dot_2,t_dot_2,l_1,l_2,A,A_2,Iax_2,Iay_2,Iaz_2,Iax_1,Iay_1,Iaz_1,Imx_1,Imy_1,Imz_1,Imx_2,Imy_2,Imz_2,m_1,m_2,g_x,g_y,g_z,Gs_1,E_1,Gs_2,E_2);
C_1_3 = C13(k_1,b_1,t_1,k_2,b_2,t_2,k_dot_1,b_dot_1,t_dot_1,k_dot_2,b_dot_2,t_dot_2,l_1,l_2,A,A_2,Iax_2,Iay_2,Iaz_2,Iax_1,Iay_1,Iaz_1,Imx_1,Imy_1,Imz_1,Imx_2,Imy_2,Imz_2,m_1,m_2,g_x,g_y,g_z,Gs_1,E_1,Gs_2,E_2);
C_1_4 = C14(k_1,b_1,t_1,k_2,b_2,t_2,k_dot_1,b_dot_1,t_dot_1,k_dot_2,b_dot_2,t_dot_2,l_1,l_2,A,A_2,Iax_2,Iay_2,Iaz_2,Iax_1,Iay_1,Iaz_1,Imx_1,Imy_1,Imz_1,Imx_2,Imy_2,Imz_2,m_1,m_2,g_x,g_y,g_z,Gs_1,E_1,Gs_2,E_2);
C_1_5 = C15(k_1,b_1,t_1,k_2,b_2,t_2,k_dot_1,b_dot_1,t_dot_1,k_dot_2,b_dot_2,t_dot_2,l_1,l_2,A,A_2,Iax_2,Iay_2,Iaz_2,Iax_1,Iay_1,Iaz_1,Imx_1,Imy_1,Imz_1,Imx_2,Imy_2,Imz_2,m_1,m_2,g_x,g_y,g_z,Gs_1,E_1,Gs_2,E_2);
C_1_6 = C16(k_1,b_1,t_1,k_2,b_2,t_2,k_dot_1,b_dot_1,t_dot_1,k_dot_2,b_dot_2,t_dot_2,l_1,l_2,A,A_2,Iax_2,Iay_2,Iaz_2,Iax_1,Iay_1,Iaz_1,Imx_1,Imy_1,Imz_1,Imx_2,Imy_2,Imz_2,m_1,m_2,g_x,g_y,g_z,Gs_1,E_1,Gs_2,E_2);

C_2_1 = C21(k_1,b_1,t_1,k_2,b_2,t_2,k_dot_1,b_dot_1,t_dot_1,k_dot_2,b_dot_2,t_dot_2,l_1,l_2,A,A_2,Iax_2,Iay_2,Iaz_2,Iax_1,Iay_1,Iaz_1,Imx_1,Imy_1,Imz_1,Imx_2,Imy_2,Imz_2,m_1,m_2,g_x,g_y,g_z,Gs_1,E_1,Gs_2,E_2);
C_2_2 = C21(k_1,b_1,t_1,k_2,b_2,t_2,k_dot_1,b_dot_1,t_dot_1,k_dot_2,b_dot_2,t_dot_2,l_1,l_2,A,A_2,Iax_2,Iay_2,Iaz_2,Iax_1,Iay_1,Iaz_1,Imx_1,Imy_1,Imz_1,Imx_2,Imy_2,Imz_2,m_1,m_2,g_x,g_y,g_z,Gs_1,E_1,Gs_2,E_2);
C_2_3 = C21(k_1,b_1,t_1,k_2,b_2,t_2,k_dot_1,b_dot_1,t_dot_1,k_dot_2,b_dot_2,t_dot_2,l_1,l_2,A,A_2,Iax_2,Iay_2,Iaz_2,Iax_1,Iay_1,Iaz_1,Imx_1,Imy_1,Imz_1,Imx_2,Imy_2,Imz_2,m_1,m_2,g_x,g_y,g_z,Gs_1,E_1,Gs_2,E_2);
C_2_4 = C26(k_1,b_1,t_1,k_2,b_2,t_2,k_dot_1,b_dot_1,t_dot_1,k_dot_2,b_dot_2,t_dot_2,l_1,l_2,A,A_2,Iax_2,Iay_2,Iaz_2,Iax_1,Iay_1,Iaz_1,Imx_1,Imy_1,Imz_1,Imx_2,Imy_2,Imz_2,m_1,m_2,g_x,g_y,g_z,Gs_1,E_1,Gs_2,E_2);
C_2_5 = C26(k_1,b_1,t_1,k_2,b_2,t_2,k_dot_1,b_dot_1,t_dot_1,k_dot_2,b_dot_2,t_dot_2,l_1,l_2,A,A_2,Iax_2,Iay_2,Iaz_2,Iax_1,Iay_1,Iaz_1,Imx_1,Imy_1,Imz_1,Imx_2,Imy_2,Imz_2,m_1,m_2,g_x,g_y,g_z,Gs_1,E_1,Gs_2,E_2);
C_2_6 = C26(k_1,b_1,t_1,k_2,b_2,t_2,k_dot_1,b_dot_1,t_dot_1,k_dot_2,b_dot_2,t_dot_2,l_1,l_2,A,A_2,Iax_2,Iay_2,Iaz_2,Iax_1,Iay_1,Iaz_1,Imx_1,Imy_1,Imz_1,Imx_2,Imy_2,Imz_2,m_1,m_2,g_x,g_y,g_z,Gs_1,E_1,Gs_2,E_2);

C_3_1 = C31(k_1,b_1,t_1,k_2,b_2,t_2,k_dot_1,b_dot_1,t_dot_1,k_dot_2,b_dot_2,t_dot_2,l_1,l_2,A,A_2,Iax_2,Iay_2,Iaz_2,Iax_1,Iay_1,Iaz_1,Imx_1,Imy_1,Imz_1,Imx_2,Imy_2,Imz_2,m_1,m_2,g_x,g_y,g_z,Gs_1,E_1,Gs_2,E_2);
C_3_2 = C32(k_1,b_1,t_1,k_2,b_2,t_2,k_dot_1,b_dot_1,t_dot_1,k_dot_2,b_dot_2,t_dot_2,l_1,l_2,A,A_2,Iax_2,Iay_2,Iaz_2,Iax_1,Iay_1,Iaz_1,Imx_1,Imy_1,Imz_1,Imx_2,Imy_2,Imz_2,m_1,m_2,g_x,g_y,g_z,Gs_1,E_1,Gs_2,E_2);
C_3_3 = C33(k_1,b_1,t_1,k_2,b_2,t_2,k_dot_1,b_dot_1,t_dot_1,k_dot_2,b_dot_2,t_dot_2,l_1,l_2,A,A_2,Iax_2,Iay_2,Iaz_2,Iax_1,Iay_1,Iaz_1,Imx_1,Imy_1,Imz_1,Imx_2,Imy_2,Imz_2,m_1,m_2,g_x,g_y,g_z,Gs_1,E_1,Gs_2,E_2);
C_3_4 =C34(k_1,b_1,t_1,k_2,b_2,t_2,k_dot_1,b_dot_1,t_dot_1,k_dot_2,b_dot_2,t_dot_2,l_1,l_2,A,A_2,Iax_2,Iay_2,Iaz_2,Iax_1,Iay_1,Iaz_1,Imx_1,Imy_1,Imz_1,Imx_2,Imy_2,Imz_2,m_1,m_2,g_x,g_y,g_z,Gs_1,E_1,Gs_2,E_2);
C_3_5 = C35(k_1,b_1,t_1,k_2,b_2,t_2,k_dot_1,b_dot_1,t_dot_1,k_dot_2,b_dot_2,t_dot_2,l_1,l_2,A,A_2,Iax_2,Iay_2,Iaz_2,Iax_1,Iay_1,Iaz_1,Imx_1,Imy_1,Imz_1,Imx_2,Imy_2,Imz_2,m_1,m_2,g_x,g_y,g_z,Gs_1,E_1,Gs_2,E_2);
C_3_6 =C36(k_1,b_1,t_1,k_2,b_2,t_2,k_dot_1,b_dot_1,t_dot_1,k_dot_2,b_dot_2,t_dot_2,l_1,l_2,A,A_2,Iax_2,Iay_2,Iaz_2,Iax_1,Iay_1,Iaz_1,Imx_1,Imy_1,Imz_1,Imx_2,Imy_2,Imz_2,m_1,m_2,g_x,g_y,g_z,Gs_1,E_1,Gs_2,E_2);

C_4_1 = C41(k_1,b_1,t_1,k_2,b_2,t_2,k_dot_1,b_dot_1,t_dot_1,k_dot_2,b_dot_2,t_dot_2,l_1,l_2,A,A_2,Iax_2,Iay_2,Iaz_2,Iax_1,Iay_1,Iaz_1,Imx_1,Imy_1,Imz_1,Imx_2,Imy_2,Imz_2,m_1,m_2,g_x,g_y,g_z,Gs_1,E_1,Gs_2,E_2);
C_4_2 = C42(k_1,b_1,t_1,k_2,b_2,t_2,k_dot_1,b_dot_1,t_dot_1,k_dot_2,b_dot_2,t_dot_2,l_1,l_2,A,A_2,Iax_2,Iay_2,Iaz_2,Iax_1,Iay_1,Iaz_1,Imx_1,Imy_1,Imz_1,Imx_2,Imy_2,Imz_2,m_1,m_2,g_x,g_y,g_z,Gs_1,E_1,Gs_2,E_2);
C_4_3 =C43(k_1,b_1,t_1,k_2,b_2,t_2,k_dot_1,b_dot_1,t_dot_1,k_dot_2,b_dot_2,t_dot_2,l_1,l_2,A,A_2,Iax_2,Iay_2,Iaz_2,Iax_1,Iay_1,Iaz_1,Imx_1,Imy_1,Imz_1,Imx_2,Imy_2,Imz_2,m_1,m_2,g_x,g_y,g_z,Gs_1,E_1,Gs_2,E_2);
C_4_4 =C44(k_1,b_1,t_1,k_2,b_2,t_2,k_dot_1,b_dot_1,t_dot_1,k_dot_2,b_dot_2,t_dot_2,l_1,l_2,A,A_2,Iax_2,Iay_2,Iaz_2,Iax_1,Iay_1,Iaz_1,Imx_1,Imy_1,Imz_1,Imx_2,Imy_2,Imz_2,m_1,m_2,g_x,g_y,g_z,Gs_1,E_1,Gs_2,E_2);
C_4_5 =C45(k_1,b_1,t_1,k_2,b_2,t_2,k_dot_1,b_dot_1,t_dot_1,k_dot_2,b_dot_2,t_dot_2,l_1,l_2,A,A_2,Iax_2,Iay_2,Iaz_2,Iax_1,Iay_1,Iaz_1,Imx_1,Imy_1,Imz_1,Imx_2,Imy_2,Imz_2,m_1,m_2,g_x,g_y,g_z,Gs_1,E_1,Gs_2,E_2);
C_4_6 =C46(k_1,b_1,t_1,k_2,b_2,t_2,k_dot_1,b_dot_1,t_dot_1,k_dot_2,b_dot_2,t_dot_2,l_1,l_2,A,A_2,Iax_2,Iay_2,Iaz_2,Iax_1,Iay_1,Iaz_1,Imx_1,Imy_1,Imz_1,Imx_2,Imy_2,Imz_2,m_1,m_2,g_x,g_y,g_z,Gs_1,E_1,Gs_2,E_2);

C_5_1 =C51(k_1,b_1,t_1,k_2,b_2,t_2,k_dot_1,b_dot_1,t_dot_1,k_dot_2,b_dot_2,t_dot_2,l_1,l_2,A,A_2,Iax_2,Iay_2,Iaz_2,Iax_1,Iay_1,Iaz_1,Imx_1,Imy_1,Imz_1,Imx_2,Imy_2,Imz_2,m_1,m_2,g_x,g_y,g_z,Gs_1,E_1,Gs_2,E_2);
C_5_2 = C52(k_1,b_1,t_1,k_2,b_2,t_2,k_dot_1,b_dot_1,t_dot_1,k_dot_2,b_dot_2,t_dot_2,l_1,l_2,A,A_2,Iax_2,Iay_2,Iaz_2,Iax_1,Iay_1,Iaz_1,Imx_1,Imy_1,Imz_1,Imx_2,Imy_2,Imz_2,m_1,m_2,g_x,g_y,g_z,Gs_1,E_1,Gs_2,E_2);
C_5_3 =C53(k_1,b_1,t_1,k_2,b_2,t_2,k_dot_1,b_dot_1,t_dot_1,k_dot_2,b_dot_2,t_dot_2,l_1,l_2,A,A_2,Iax_2,Iay_2,Iaz_2,Iax_1,Iay_1,Iaz_1,Imx_1,Imy_1,Imz_1,Imx_2,Imy_2,Imz_2,m_1,m_2,g_x,g_y,g_z,Gs_1,E_1,Gs_2,E_2);
C_5_4 =C54(k_1,b_1,t_1,k_2,b_2,t_2,k_dot_1,b_dot_1,t_dot_1,k_dot_2,b_dot_2,t_dot_2,l_1,l_2,A,A_2,Iax_2,Iay_2,Iaz_2,Iax_1,Iay_1,Iaz_1,Imx_1,Imy_1,Imz_1,Imx_2,Imy_2,Imz_2,m_1,m_2,g_x,g_y,g_z,Gs_1,E_1,Gs_2,E_2);
C_5_5 =C55(k_1,b_1,t_1,k_2,b_2,t_2,k_dot_1,b_dot_1,t_dot_1,k_dot_2,b_dot_2,t_dot_2,l_1,l_2,A,A_2,Iax_2,Iay_2,Iaz_2,Iax_1,Iay_1,Iaz_1,Imx_1,Imy_1,Imz_1,Imx_2,Imy_2,Imz_2,m_1,m_2,g_x,g_y,g_z,Gs_1,E_1,Gs_2,E_2);
C_5_6 =C56(k_1,b_1,t_1,k_2,b_2,t_2,k_dot_1,b_dot_1,t_dot_1,k_dot_2,b_dot_2,t_dot_2,l_1,l_2,A,A_2,Iax_2,Iay_2,Iaz_2,Iax_1,Iay_1,Iaz_1,Imx_1,Imy_1,Imz_1,Imx_2,Imy_2,Imz_2,m_1,m_2,g_x,g_y,g_z,Gs_1,E_1,Gs_2,E_2);

C_6_1 =C61(k_1,b_1,t_1,k_2,b_2,t_2,k_dot_1,b_dot_1,t_dot_1,k_dot_2,b_dot_2,t_dot_2,l_1,l_2,A,A_2,Iax_2,Iay_2,Iaz_2,Iax_1,Iay_1,Iaz_1,Imx_1,Imy_1,Imz_1,Imx_2,Imy_2,Imz_2,m_1,m_2,g_x,g_y,g_z,Gs_1,E_1,Gs_2,E_2);
C_6_2 = C62(k_1,b_1,t_1,k_2,b_2,t_2,k_dot_1,b_dot_1,t_dot_1,k_dot_2,b_dot_2,t_dot_2,l_1,l_2,A,A_2,Iax_2,Iay_2,Iaz_2,Iax_1,Iay_1,Iaz_1,Imx_1,Imy_1,Imz_1,Imx_2,Imy_2,Imz_2,m_1,m_2,g_x,g_y,g_z,Gs_1,E_1,Gs_2,E_2);
C_6_3 =C63(k_1,b_1,t_1,k_2,b_2,t_2,k_dot_1,b_dot_1,t_dot_1,k_dot_2,b_dot_2,t_dot_2,l_1,l_2,A,A_2,Iax_2,Iay_2,Iaz_2,Iax_1,Iay_1,Iaz_1,Imx_1,Imy_1,Imz_1,Imx_2,Imy_2,Imz_2,m_1,m_2,g_x,g_y,g_z,Gs_1,E_1,Gs_2,E_2);
C_6_4 =C64(k_1,b_1,t_1,k_2,b_2,t_2,k_dot_1,b_dot_1,t_dot_1,k_dot_2,b_dot_2,t_dot_2,l_1,l_2,A,A_2,Iax_2,Iay_2,Iaz_2,Iax_1,Iay_1,Iaz_1,Imx_1,Imy_1,Imz_1,Imx_2,Imy_2,Imz_2,m_1,m_2,g_x,g_y,g_z,Gs_1,E_1,Gs_2,E_2);
C_6_5 =C65(k_1,b_1,t_1,k_2,b_2,t_2,k_dot_1,b_dot_1,t_dot_1,k_dot_2,b_dot_2,t_dot_2,l_1,l_2,A,A_2,Iax_2,Iay_2,Iaz_2,Iax_1,Iay_1,Iaz_1,Imx_1,Imy_1,Imz_1,Imx_2,Imy_2,Imz_2,m_1,m_2,g_x,g_y,g_z,Gs_1,E_1,Gs_2,E_2);
C_6_6 =C66(k_1,b_1,t_1,k_2,b_2,t_2,k_dot_1,b_dot_1,t_dot_1,k_dot_2,b_dot_2,t_dot_2,l_1,l_2,A,A_2,Iax_2,Iay_2,Iaz_2,Iax_1,Iay_1,Iaz_1,Imx_1,Imy_1,Imz_1,Imx_2,Imy_2,Imz_2,m_1,m_2,g_x,g_y,g_z,Gs_1,E_1,Gs_2,E_2);

C_n = [ C_1_1,C_1_2,C_1_3,C_1_4,C_1_5,C_1_6;
        C_2_1,C_2_2,C_2_3,C_2_4,C_2_5,C_2_6;
        C_3_1,C_3_2,C_3_3,C_3_4,C_3_5,C_3_6;
        C_4_1,C_4_2,C_4_3,C_4_4,C_4_5,C_4_6;
        C_5_1,C_5_2,C_5_3,C_5_4,C_5_5,C_5_6;
        C_6_1,C_6_2,C_6_3,C_6_4,C_6_5,C_6_6;
      ];
 J1_n= J_1(b_1,k_1,l_1,t_1);
 J2_n= J_2(b_1,b_2,k_1,k_2,l_1,l_2,t_1,t_2);
 B_n=B(k_1,b_1,t_1,k_2,b_2,t_2,k_dot_1,b_dot_1,t_dot_1,k_dot_2,b_dot_2,t_dot_2,l_1,l_2,A,A_2,Iax_2,Iay_2,Iaz_2,Iax_1,Iay_1,Iaz_1,Imx_1,Imy_1,Imz_1,Imx_2,Imy_2,Imz_2,m_1,m_2,g_x,g_y,g_z,Gs_1,E_1,Gs_2,E_2);
 G_n =G(k_1,b_1,t_1,k_2,b_2,t_2,k_dot_1,b_dot_1,t_dot_1,k_dot_2,b_dot_2,t_dot_2,l_1,l_2,A,A_2,Iax_2,Iay_2,Iaz_2,Iax_1,Iay_1,Iaz_1,Imx_1,Imy_1,Imz_1,Imx_2,Imy_2,Imz_2,m_1,m_2,g_x,g_y,g_z,Gs_1,E_1,Gs_2,E_2);
D_n = D;

== matlab function dyn_control/Subsystem/MATLAB Function ==
  data: u input; tensions output
function tensions = fcn(u)
    control_k_1 = u(1);
    control_b_1 = u(2);
    control_t_1 = u(3);
    control_k_2 = u(4);
    control_b_2 = u(5);
    control_t_2 = u(6);

    if control_k_2>= 0
        T_1 = control_k_2;
        T_2 = 0;
    else
        T_2 = control_k_2;
        T_1 = 0;
    end
    if control_b_2 >= 0
        T_3 = control_b_2;
        T_4 = 0;
    else
        T_4 = control_b_2;
        T_3 = 0;
    end
    if control_t_2>0
        T_5 = control_t_2;
    else 
        T_5 = 0;
    end
    tensions = [T_1 T_2 T_3 ,T_4 , T_5];

== matlab function dyn_control/Subsystem1/MATLAB Function1 ==
  data: q input; x output; l_1 input; l_2 input; y output; z output; roll output; pitch output; yaw output
function [x , y , z , roll , pitch ,yaw ] = fcn(q,l_1,l_2)
    k_1 = q(1);
    b_1 = q(2);
    t_1 = q(3);
    k_2 = q(4);
    b_2 = q(5);
    t_2 = q(6);
    T1 = T_1(b_1,k_1,l_1,t_1);
    T2 = T_2(b_2,k_2,l_2,t_2);

    T_01 = T1;
    tw = T1 * T2;

    x = tw(1,4) ;
    y = tw(2,4) ;
    z = tw(3,4) ;
    roll = tw(3,2) ;
    pitch = tw(1,3) ;
    yaw = tw(2,1) ;
